simulink model "elevator"  (R2020a)
settings: Solver=VariableStepAuto  StartTime=0.0  StopTime=inf  RelTol=1e-3
PreLoadFcn:
  | slplc.api.loadDataTypes;
undefined symbols (not defined in the file): BOOL, DINT, INT, slplc
libraries: simulink x1
(part 2 of 38)

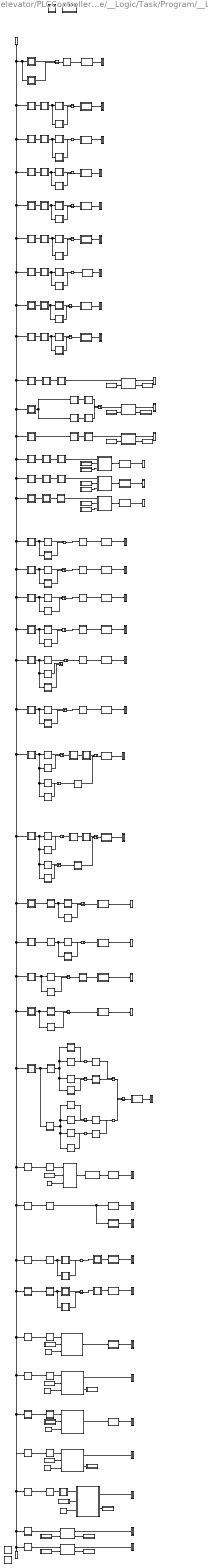
== system elevator/PLCControllerSuite/__Logic/Task/Program/__Logic ==
  note: Increment motor speed by 0.01
  note: Latch motor increase procedure
  note: Initiate motor speed decrease after appropriate sensor is triggered
  note: Trigger motor to increase speed after delay
  note: Indicates when the last direction traveled was up.
  note: Checking for appropriate floor sensor to initiate slow down.
  note: Motor is ON
  note: Motor direction is down
  note: Motor direction is up
  note: Request floor 1
  note: Start/Stop
  note: Request floor 2
  note: Request floor 3
  note: Request elevator to go to floor 2
  note: Memory, to control motor to go down.
  note: Request elevator to go to floor 1
  note: Memory, to control motor to go up.
  note: Request elevator to go to floor 3
  note: Tracck Floor 1
  note: Tracck Floor 2
  note: Tracck Floor 3
  note: Store current position if floor 1
  note: Store current position if floor 2
  note: Store current position if floor 3
  note: TracK Elevator going away or towards Floor 3
  note: TracK Elevator going away or towards Floor 2
  note: TracK Elevator going away or towards Floor 1
  note: Latch motor decrease procedure
  note: Decriment motor speed by 0.01
  note: Set motor speed to 0 when at appropriate floor
  note: Increase speed if less than or equal MAXVEL
  note: Decrease speed if greater than ZERO
  note: Send motor speed out
  note: Send motor speed out
  ADD : Subsystem  Priority=274  TreatAsAtomicUnit=on  mask{PLCBlockType=ADD, PLCPOUType=stdFC}
      mask Help: web([docroot '/plccoder/ref/add' '.html']);
      mask DialogControl PLCBlockTitle Prompt: Add (ADD)
      mask DialogControl PLCBlockDesc Prompt: Add Source A and Source B.
      mask Display: disp('ADD');
  Add Rungs : Subsystem  DisableCoverage=on  TreatAsAtomicUnit=on  mask{PLCRungNumberToAdd=1, PLCBlockType=AddRungs}
      mask prompts: PLCRungNumberToAdd "Rung Number:"
      mask Help: web([docroot '/plccoder/ref/addrungs' '.html']);
      mask DialogControl PLCAddRungs Prompt: Add Rungs
      mask DialogControl PLCRungAddButton Prompt: Add
      mask DialogControl PLCRungAddButton Callback: slplc.callbacks.addLadderRungs(gcb);
      mask Display: disp(sprintf(['Add' newline 'Rungs']));
  Add Single Rung : Subsystem  DisableCoverage=on  TreatAsAtomicUnit=on  mask{PLCRungNumberToAdd=1, PLCBlockType=AddSingleRung}
      settings: OpenFcn=slplc.callbacks.addLadderRungs(gcb);
      mask Help: web([docroot '/plccoder/ref/addsinglerung' '.html']);
      mask DialogControl PLCAddRung Prompt: Add Single Rung
      mask Display: disp(sprintf(['Add' newline '1 Rung']));
  Constant : Constant  Priority=236  Value=0
  Constant1 : Constant  Priority=273  Value=0.01
  Constant2 : Constant  Priority=287  Value=0.01
  Constant3 : Constant  Priority=295  Value=0
  Constant4 : Constant  Priority=266  Value=24
  Constant5 : Constant  Priority=280  Value=0.01
  EQU : Subsystem  Priority=109  TreatAsAtomicUnit=on  mask{PLCBlockType=EQU, PLCPOUType=stdFC}
      mask Help: web([docroot '/plccoder/ref/equ' '.html']);
      mask DialogControl PLCBlockTitle Prompt: Equal To (EQU)
      mask DialogControl PLCBlockDesc Prompt: Test whether Source A is equal to Source B.
      mask Display: disp('EQU');
  EQU1 : Subsystem  Priority=101  TreatAsAtomicUnit=on  mask{PLCBlockType=EQU, PLCPOUType=stdFC}
      mask Help: web([docroot '/plccoder/ref/equ' '.html']);
      mask DialogControl PLCBlockTitle Prompt: Equal To (EQU)
      mask DialogControl PLCBlockDesc Prompt: Test whether Source A is equal to Source B.
      mask Display: disp('EQU');
  EQU2 : Subsystem  Priority=93  TreatAsAtomicUnit=on  mask{PLCBlockType=EQU, PLCPOUType=stdFC}
      mask Help: web([docroot '/plccoder/ref/equ' '.html']);
      mask DialogControl PLCBlockTitle Prompt: Equal To (EQU)
      mask DialogControl PLCBlockDesc Prompt: Test whether Source A is equal to Source B.
      mask Display: disp('EQU');
  EQU3 : Subsystem  Priority=237  TreatAsAtomicUnit=on  mask{PLCBlockType=EQU, PLCPOUType=stdFC}
      mask Help: web([docroot '/plccoder/ref/equ' '.html']);
      mask DialogControl PLCBlockTitle Prompt: Equal To (EQU)
      mask DialogControl PLCBlockDesc Prompt: Test whether Source A is equal to Source B.
      mask Display: disp('EQU');
  GRT : Subsystem  Priority=281  TreatAsAtomicUnit=on  mask{PLCBlockType=GRT, PLCPOUType=stdFC}
      mask Help: web([docroot '/plccoder/ref/grt' '.html']);
      mask DialogControl PLCBlockTitle Prompt: Greater Than (GRT)
      mask DialogControl PLCBlockDesc Prompt: Test whether Source A is greater than Source B.
      mask Display: disp('GRT');
  Junction : Subsystem  Priority=186  DisableCoverage=on  TreatAsAtomicUnit=on  mask{PLCBlockType=Junction, PLCPOUType=BranchJunction}
      mask Help: web([docroot '/plccoder/ref/junction' '.html']);
      mask DialogControl PLCBlockTitle Prompt: Rung Merge Point
      mask DialogControl PLCBlockDesc Prompt: This is the ladder diagram rung merge point.
  Junction1 : Subsystem  Priority=115  DisableCoverage=on  TreatAsAtomicUnit=on  mask{PLCBlockType=Junction, PLCPOUType=BranchJunction}
      mask Help: web([docroot '/plccoder/ref/junction' '.html']);
      mask DialogControl PLCBlockTitle Prompt: Rung Merge Point
      mask DialogControl PLCBlockDesc Prompt: This is the ladder diagram rung merge point.
  Junction10 : Subsystem  Priority=164  DisableCoverage=on  TreatAsAtomicUnit=on  mask{PLCBlockType=Junction, PLCPOUType=BranchJunction}
      mask Help: web([docroot '/plccoder/ref/junction' '.html']);
      mask DialogControl PLCBlockTitle Prompt: Rung Merge Point
      mask DialogControl PLCBlockDesc Prompt: This is the ladder diagram rung merge point.
  Junction11 : Subsystem  Priority=179  DisableCoverage=on  TreatAsAtomicUnit=on  mask{PLCBlockType=Junction, PLCPOUType=BranchJunction}
      mask Help: web([docroot '/plccoder/ref/junction' '.html']);
      mask DialogControl PLCBlockTitle Prompt: Rung Merge Point
      mask DialogControl PLCBlockDesc Prompt: This is the ladder diagram rung merge point.
  Junction12 : Subsystem  Priority=172  DisableCoverage=on  TreatAsAtomicUnit=on  mask{PLCBlockType=Junction, PLCPOUType=BranchJunction}
      mask Help: web([docroot '/plccoder/ref/junction' '.html']);
      mask DialogControl PLCBlockTitle Prompt: Rung Merge Point
      mask DialogControl PLCBlockDesc Prompt: This is the ladder diagram rung merge point.
  Junction13 : Subsystem  Priority=177  DisableCoverage=on  TreatAsAtomicUnit=on  mask{PLCBlockType=Junction, PLCPOUType=BranchJunction}
      mask Help: web([docroot '/plccoder/ref/junction' '.html']);
      mask DialogControl PLCBlockTitle Prompt: Rung Merge Point
      mask DialogControl PLCBlockDesc Prompt: This is the ladder diagram rung merge point.
  Junction14 : Subsystem  Priority=227  DisableCoverage=on  TreatAsAtomicUnit=on  mask{PLCBlockType=Junction, PLCPOUType=BranchJunction}
      mask Help: web([docroot '/plccoder/ref/junction' '.html']);
      mask DialogControl PLCBlockTitle Prompt: Rung Merge Point
      mask DialogControl PLCBlockDesc Prompt: This is the ladder diagram rung merge point.
  Junction15 : Subsystem  Priority=223  DisableCoverage=on  TreatAsAtomicUnit=on  mask{PLCBlockType=Junction, PLCPOUType=BranchJunction}
      mask Help: web([docroot '/plccoder/ref/junction' '.html']);
      mask DialogControl PLCBlockTitle Prompt: Rung Merge Point
      mask DialogControl PLCBlockDesc Prompt: This is the ladder diagram rung merge point.
  Junction16 : Subsystem  Priority=219  DisableCoverage=on  TreatAsAtomicUnit=on  mask{PLCBlockType=Junction, PLCPOUType=BranchJunction}
      mask Help: web([docroot '/plccoder/ref/junction' '.html']);
      mask DialogControl PLCBlockTitle Prompt: Rung Merge Point
      mask DialogControl PLCBlockDesc Prompt: This is the ladder diagram rung merge point.
  Junction17 : Subsystem  Priority=229  DisableCoverage=on  TreatAsAtomicUnit=on  mask{PLCBlockType=Junction, PLCPOUType=BranchJunction}
      mask Help: web([docroot '/plccoder/ref/junction' '.html']);
      mask DialogControl PLCBlockTitle Prompt: Rung Merge Point
      mask DialogControl PLCBlockDesc Prompt: This is the ladder diagram rung merge point.
  Junction18 : Subsystem  Priority=193  DisableCoverage=on  TreatAsAtomicUnit=on  mask{PLCBlockType=Junction, PLCPOUType=BranchJunction}
      mask Help: web([docroot '/plccoder/ref/junction' '.html']);
      mask DialogControl PLCBlockTitle Prompt: Rung Merge Point
      mask DialogControl PLCBlockDesc Prompt: This is the ladder diagram rung merge point.
  Junction19 : Subsystem  Priority=213  DisableCoverage=on  TreatAsAtomicUnit=on  mask{PLCBlockType=Junction, PLCPOUType=BranchJunction}
      mask Help: web([docroot '/plccoder/ref/junction' '.html']);
      mask DialogControl PLCBlockTitle Prompt: Rung Merge Point
      mask DialogControl PLCBlockDesc Prompt: This is the ladder diagram rung merge point.
  Junction2 : Subsystem  Priority=122  DisableCoverage=on  TreatAsAtomicUnit=on  mask{PLCBlockType=Junction, PLCPOUType=BranchJunction}
      mask Help: web([docroot '/plccoder/ref/junction' '.html']);
      mask DialogControl PLCBlockTitle Prompt: Rung Merge Point
      mask DialogControl PLCBlockDesc Prompt: This is the ladder diagram rung merge point.
  Junction20 : Subsystem  Priority=4  DisableCoverage=on  TreatAsAtomicUnit=on  mask{PLCBlockType=Junction, PLCPOUType=BranchJunction}
      mask Help: web([docroot '/plccoder/ref/junction' '.html']);
      mask DialogControl PLCBlockTitle Prompt: Rung Merge Point
      mask DialogControl PLCBlockDesc Prompt: This is the ladder diagram rung merge point.
  Junction21 : Subsystem  Priority=217  DisableCoverage=on  TreatAsAtomicUnit=on  mask{PLCBlockType=Junction, PLCPOUType=BranchJunction}
      mask Help: web([docroot '/plccoder/ref/junction' '.html']);
      mask DialogControl PLCBlockTitle Prompt: Rung Merge Point
      mask DialogControl PLCBlockDesc Prompt: This is the ladder diagram rung merge point.
  Junction22 : Subsystem  Priority=19  DisableCoverage=on  TreatAsAtomicUnit=on  mask{PLCBlockType=Junction, PLCPOUType=BranchJunction}
      mask Help: web([docroot '/plccoder/ref/junction' '.html']);
      mask DialogControl PLCBlockTitle Prompt: Rung Merge Point
      mask DialogControl PLCBlockDesc Prompt: This is the ladder diagram rung merge point.
  Junction23 : Subsystem  Priority=26  DisableCoverage=on  TreatAsAtomicUnit=on  mask{PLCBlockType=Junction, PLCPOUType=BranchJunction}
      mask Help: web([docroot '/plccoder/ref/junction' '.html']);
      mask DialogControl PLCBlockTitle Prompt: Rung Merge Point
      mask DialogControl PLCBlockDesc Prompt: This is the ladder diagram rung merge point.
  Junction24 : Subsystem  Priority=76  DisableCoverage=on  TreatAsAtomicUnit=on  mask{PLCBlockType=Junction, PLCPOUType=BranchJunction}
      mask Help: web([docroot '/plccoder/ref/junction' '.html']);
      mask DialogControl PLCBlockTitle Prompt: Rung Merge Point
      mask DialogControl PLCBlockDesc Prompt: This is the ladder diagram rung merge point.
  Junction25 : Subsystem  Priority=54  DisableCoverage=on  TreatAsAtomicUnit=on  mask{PLCBlockType=Junction, PLCPOUType=BranchJunction}
      mask Help: web([docroot '/plccoder/ref/junction' '.html']);
      mask DialogControl PLCBlockTitle Prompt: Rung Merge Point
      mask DialogControl PLCBlockDesc Prompt: This is the ladder diagram rung merge point.
  Junction26 : Subsystem  Priority=40  DisableCoverage=on  TreatAsAtomicUnit=on  mask{PLCBlockType=Junction, PLCPOUType=BranchJunction}
      mask Help: web([docroot '/plccoder/ref/junction' '.html']);
      mask DialogControl PLCBlockTitle Prompt: Rung Merge Point
      mask DialogControl PLCBlockDesc Prompt: This is the ladder diagram rung merge point.
  Junction27 : Subsystem  Priority=61  DisableCoverage=on  TreatAsAtomicUnit=on  mask{PLCBlockType=Junction, PLCPOUType=BranchJunction}
      mask Help: web([docroot '/plccoder/ref/junction' '.html']);
      mask DialogControl PLCBlockTitle Prompt: Rung Merge Point
      mask DialogControl PLCBlockDesc Prompt: This is the ladder diagram rung merge point.
  Junction28 : Subsystem  Priority=47  DisableCoverage=on  TreatAsAtomicUnit=on  mask{PLCBlockType=Junction, PLCPOUType=BranchJunction}
      mask Help: web([docroot '/plccoder/ref/junction' '.html']);
      mask DialogControl PLCBlockTitle Prompt: Rung Merge Point
      mask DialogControl PLCBlockDesc Prompt: This is the ladder diagram rung merge point.
  Junction29 : Subsystem  Priority=206  DisableCoverage=on  TreatAsAtomicUnit=on  mask{PLCBlockType=Junction, PLCPOUType=BranchJunction}
      mask Help: web([docroot '/plccoder/ref/junction' '.html']);
      mask DialogControl PLCBlockTitle Prompt: Rung Merge Point
      mask DialogControl PLCBlockDesc Prompt: This is the ladder diagram rung merge point.
  Junction3 : Subsystem  Priority=129  DisableCoverage=on  TreatAsAtomicUnit=on  mask{PLCBlockType=Junction, PLCPOUType=BranchJunction}
      mask Help: web([docroot '/plccoder/ref/junction' '.html']);
      mask DialogControl PLCBlockTitle Prompt: Rung Merge Point
      mask DialogControl PLCBlockDesc Prompt: This is the ladder diagram rung merge point.
  Junction30 : Subsystem  Priority=230  DisableCoverage=on  TreatAsAtomicUnit=on  mask{PLCBlockType=Junction, PLCPOUType=BranchJunction}
      mask Help: web([docroot '/plccoder/ref/junction' '.html']);
      mask DialogControl PLCBlockTitle Prompt: Rung Merge Point
      mask DialogControl PLCBlockDesc Prompt: This is the ladder diagram rung merge point.
  Junction31 : Subsystem  Priority=199  DisableCoverage=on  TreatAsAtomicUnit=on  mask{PLCBlockType=Junction, PLCPOUType=BranchJunction}
      mask Help: web([docroot '/plccoder/ref/junction' '.html']);
      mask DialogControl PLCBlockTitle Prompt: Rung Merge Point
      mask DialogControl PLCBlockDesc Prompt: This is the ladder diagram rung merge point.
  Junction32 : Subsystem  Priority=33  DisableCoverage=on  TreatAsAtomicUnit=on  mask{PLCBlockType=Junction, PLCPOUType=BranchJunction}
      mask Help: web([docroot '/plccoder/ref/junction' '.html']);
      mask DialogControl PLCBlockTitle Prompt: Rung Merge Point
      mask DialogControl PLCBlockDesc Prompt: This is the ladder diagram rung merge point.
  Junction33 : Subsystem  Priority=12  DisableCoverage=on  TreatAsAtomicUnit=on  mask{PLCBlockType=Junction, PLCPOUType=BranchJunction}
      mask Help: web([docroot '/plccoder/ref/junction' '.html']);
      mask DialogControl PLCBlockTitle Prompt: Rung Merge Point
      mask DialogControl PLCBlockDesc Prompt: This is the ladder diagram rung merge point.
  Junction34 : Subsystem  Priority=251  DisableCoverage=on  TreatAsAtomicUnit=on  mask{PLCBlockType=Junction, PLCPOUType=BranchJunction}
      mask Help: web([docroot '/plccoder/ref/junction' '.html']);
      mask DialogControl PLCBlockTitle Prompt: Rung Merge Point
      mask DialogControl PLCBlockDesc Prompt: This is the ladder diagram rung merge point.
  Junction35 : Subsystem  Priority=259  DisableCoverage=on  TreatAsAtomicUnit=on  mask{PLCBlockType=Junction, PLCPOUType=BranchJunction}
      mask Help: web([docroot '/plccoder/ref/junction' '.html']);
      mask DialogControl PLCBlockTitle Prompt: Rung Merge Point
      mask DialogControl PLCBlockDesc Prompt: This is the ladder diagram rung merge point.
  Junction4 : Subsystem  Priority=136  DisableCoverage=on  TreatAsAtomicUnit=on  mask{PLCBlockType=Junction, PLCPOUType=BranchJunction}
      mask Help: web([docroot '/plccoder/ref/junction' '.html']);
      mask DialogControl PLCBlockTitle Prompt: Rung Merge Point
      mask DialogControl PLCBlockDesc Prompt: This is the ladder diagram rung merge point.
  Junction5 : Subsystem  Priority=145  DisableCoverage=on  TreatAsAtomicUnit=on  mask{PLCBlockType=Junction, PLCPOUType=BranchJunction}
      mask Help: web([docroot '/plccoder/ref/junction' '.html']);
      mask DialogControl PLCBlockTitle Prompt: Rung Merge Point
      mask DialogControl PLCBlockDesc Prompt: This is the ladder diagram rung merge point.
  Junction6 : Subsystem  Priority=144  DisableCoverage=on  TreatAsAtomicUnit=on  mask{PLCBlockType=Junction, PLCPOUType=BranchJunction}
      mask Help: web([docroot '/plccoder/ref/junction' '.html']);
      mask DialogControl PLCBlockTitle Prompt: Rung Merge Point
      mask DialogControl PLCBlockDesc Prompt: This is the ladder diagram rung merge point.
  Junction7 : Subsystem  Priority=152  DisableCoverage=on  TreatAsAtomicUnit=on  mask{PLCBlockType=Junction, PLCPOUType=BranchJunction}
      mask Help: web([docroot '/plccoder/ref/junction' '.html']);
      mask DialogControl PLCBlockTitle Prompt: Rung Merge Point
      mask DialogControl PLCBlockDesc Prompt: This is the ladder diagram rung merge point.
  Junction8 : Subsystem  Priority=159  DisableCoverage=on  TreatAsAtomicUnit=on  mask{PLCBlockType=Junction, PLCPOUType=BranchJunction}
      mask Help: web([docroot '/plccoder/ref/junction' '.html']);
      mask DialogControl PLCBlockTitle Prompt: Rung Merge Point
      mask DialogControl PLCBlockDesc Prompt: This is the ladder diagram rung merge point.
  Junction9 : Subsystem  Priority=166  DisableCoverage=on  TreatAsAtomicUnit=on  mask{PLCBlockType=Junction, PLCPOUType=BranchJunction}
      mask Help: web([docroot '/plccoder/ref/junction' '.html']);
      mask DialogControl PLCBlockTitle Prompt: Rung Merge Point
      mask DialogControl PLCBlockDesc Prompt: This is the ladder diagram rung merge point.
  LEQ : Subsystem  Priority=267  TreatAsAtomicUnit=on  mask{PLCBlockType=LEQ, PLCPOUType=stdFC}
      mask Help: web([docroot '/plccoder/ref/leq' '.html']);
      mask DialogControl PLCBlockTitle Prompt: Less Than or Equal To (LEQ)
      mask DialogControl PLCBlockDesc Prompt: Test whether Source A is less than or equal to Source B.
      mask Display: disp('LEQ');
  MOV : Subsystem  Priority=301  TreatAsAtomicUnit=on  mask{PLCBlockType=MOV, PLCPOUType=stdFC}
      mask Help: web([docroot '/plccoder/ref/mov' '.html']);
      mask DialogControl PLCBlockTitle Prompt: Move (MOV)
      mask DialogControl PLCBlockDesc Prompt: Move a copy of the Source to the Destination. The Source remains unchanged.
      mask Display: disp('MOV');
  MOV1 : Subsystem  Priority=85  TreatAsAtomicUnit=on  mask{PLCBlockType=MOV, PLCPOUType=stdFC}
      mask Help: web([docroot '/plccoder/ref/mov' '.html']);
      mask DialogControl PLCBlockTitle Prompt: Move (MOV)
      mask DialogControl PLCBlockDesc Prompt: Move a copy of the Source to the Destination. The Source remains unchanged.
      mask Display: disp('MOV');
  MOV2 : Subsystem  Priority=78  TreatAsAtomicUnit=on  mask{PLCBlockType=MOV, PLCPOUType=stdFC}
      mask Help: web([docroot '/plccoder/ref/mov' '.html']);
      mask DialogControl PLCBlockTitle Prompt: Move (MOV)
      mask DialogControl PLCBlockDesc Prompt: Move a copy of the Source to the Destination. The Source remains unchanged.
      mask Display: disp('MOV');
  MOV3 : Subsystem  Priority=68  TreatAsAtomicUnit=on  mask{PLCBlockType=MOV, PLCPOUType=stdFC}
      mask Help: web([docroot '/plccoder/ref/mov' '.html']);
      mask DialogControl PLCBlockTitle Prompt: Move (MOV)
      mask DialogControl PLCBlockDesc Prompt: Move a copy of the Source to the Destination. The Source remains unchanged.
      mask Display: disp('MOV');
  MOV4 : Subsystem  Priority=306  TreatAsAtomicUnit=on  mask{PLCBlockType=MOV, PLCPOUType=stdFC}
      mask Help: web([docroot '/plccoder/ref/mov' '.html']);
      mask DialogControl PLCBlockTitle Prompt: Move (MOV)
      mask DialogControl PLCBlockDesc Prompt: Move a copy of the Source to the Destination. The Source remains unchanged.
      mask Display: disp('MOV');
  MUL : Subsystem  Priority=296  TreatAsAtomicUnit=on  mask{PLCBlockType=MUL, PLCPOUType=stdFC}
      mask Help: web([docroot '/plccoder/ref/mul' '.html']);
      mask DialogControl PLCBlockTitle Prompt: Multiply (MUL)
      mask DialogControl PLCBlockDesc Prompt: Multiply Source A with Source B.
      mask Display: disp('MUL');
  OTE : Subsystem  Priority=6  TreatAsAtomicUnit=on  mask{PLCOperandTag=StartHold, PLCBlockType=OTE, PLCPOUType=Coil, PLCOperandExpression=xxx_PLC_VAR_StartHold}
      mask prompts: PLCOperandTag "Operand Tag:"
      mask init:
      | slplc.callbacks.initInstruction(gcb);
      settings: AttributesFormatString=%<PLCOperandTag>
      mask Help: web([docroot '/plccoder/ref/ote' '.html']);
      mask DialogControl PLCBlockTitle Prompt: Output Energize (OTE)
  OTE1 : Subsystem  Priority=117  TreatAsAtomicUnit=on  mask{PLCOperandTag=F1PBHold, PLCBlockType=OTE, PLCPOUType=Coil, PLCOperandExpression=xxx_PLC_VAR_F1PBHold}
      mask prompts: PLCOperandTag "Operand Tag:"
      mask init:
      | slplc.callbacks.initInstruction(gcb);
      settings: AttributesFormatString=%<PLCOperandTag>
      mask Help: web([docroot '/plccoder/ref/ote' '.html']);
      mask DialogControl PLCBlockTitle Prompt: Output Energize (OTE)
  OTE10 : Subsystem  Priority=180  TreatAsAtomicUnit=on  mask{PLCOperandTag=MemoryGoDown, PLCBlockType=OTE, PLCPOUType=Coil, PLCOperandExpression=xxx_PLC_VAR_MemoryGoDown}
      mask prompts: PLCOperandTag "Operand Tag:"
      mask init:
      | slplc.callbacks.initInstruction(gcb);
      settings: AttributesFormatString=%<PLCOperandTag>
      mask Help: web([docroot '/plccoder/ref/ote' '.html']);
      mask DialogControl PLCBlockTitle Prompt: Output Energize (OTE)
  OTE11 : Subsystem  Priority=239  TreatAsAtomicUnit=on  mask{PLCOperandTag=RMPUPTRG, PLCBlockType=OTE, PLCPOUType=Coil, PLCOperandExpression=xxx_PLC_VAR_RMPUPTRG}
      mask prompts: PLCOperandTag "Operand Tag:"
      mask init:
      | slplc.callbacks.initInstruction(gcb);
      settings: AttributesFormatString=%<PLCOperandTag>
      mask Help: web([docroot '/plccoder/ref/ote' '.html']);
      mask DialogControl PLCBlockTitle Prompt: Output Energize (OTE)
  OTE12 : Subsystem  Priority=253  TreatAsAtomicUnit=on  mask{PLCOperandTag=RMPUP, PLCBlockType=OTE, PLCPOUType=Coil, PLCOperandExpression=xxx_PLC_VAR_RMPUP}
      mask prompts: PLCOperandTag "Operand Tag:"
      mask init:
      | slplc.callbacks.initInstruction(gcb);
      settings: AttributesFormatString=%<PLCOperandTag>
      mask Help: web([docroot '/plccoder/ref/ote' '.html']);
      mask DialogControl PLCBlockTitle Prompt: Output Energize (OTE)
  OTE13 : Subsystem  Priority=261  TreatAsAtomicUnit=on  mask{PLCOperandTag=RMPDN, PLCBlockType=OTE, PLCPOUType=Coil, PLCOperandExpression=xxx_PLC_VAR_RMPDN}
      mask prompts: PLCOperandTag "Operand Tag:"
      mask init:
      | slplc.callbacks.initInstruction(gcb);
      settings: AttributesFormatString=%<PLCOperandTag>
      mask Help: web([docroot '/plccoder/ref/ote' '.html']);
      mask DialogControl PLCBlockTitle Prompt: Output Energize (OTE)
  OTE14 : Subsystem  Priority=243  TreatAsAtomicUnit=on  mask{PLCOperandTag=RMPUPKIL, PLCBlockType=OTE, PLCPOUType=Coil, PLCOperandExpression=xxx_PLC_VAR_RMPUPKIL}
      mask prompts: PLCOperandTag "Operand Tag:"
      mask init:
      | slplc.callbacks.initInstruction(gcb);
      settings: AttributesFormatString=%<PLCOperandTag>
      mask Help: web([docroot '/plccoder/ref/ote' '.html']);
      mask DialogControl PLCBlockTitle Prompt: Output Energize (OTE)
  OTE15 : Subsystem  Priority=62  TreatAsAtomicUnit=on  mask{PLCOperandTag=TempS1HUp, PLCBlockType=OTE, PLCPOUType=Coil, PLCOperandExpression=xxx_PLC_VAR_TempS1HUp}
      mask prompts: PLCOperandTag "Operand Tag:"
      mask init:
      | slplc.callbacks.initInstruction(gcb);
      settings: AttributesFormatString=%<PLCOperandTag>
      mask Help: web([docroot '/plccoder/ref/ote' '.html']);
      mask DialogControl PLCBlockTitle Prompt: Output Energize (OTE)
  OTE16 : Subsystem  Priority=48  TreatAsAtomicUnit=on  mask{PLCOperandTag=TempS2LUp, PLCBlockType=OTE, PLCPOUType=Coil, PLCOperandExpression=xxx_PLC_VAR_TempS2LUp}
      mask prompts: PLCOperandTag "Operand Tag:"
      mask init:
      | slplc.callbacks.initInstruction(gcb);
      settings: AttributesFormatString=%<PLCOperandTag>
      mask Help: web([docroot '/plccoder/ref/ote' '.html']);
      mask DialogControl PLCBlockTitle Prompt: Output Energize (OTE)
  OTE17 : Subsystem  Priority=20  TreatAsAtomicUnit=on  mask{PLCOperandTag=TempS3LUp, PLCBlockType=OTE, PLCPOUType=Coil, PLCOperandExpression=xxx_PLC_VAR_TempS3LUp}
      mask prompts: PLCOperandTag "Operand Tag:"
      mask init:
      | slplc.callbacks.initInstruction(gcb);
      settings: AttributesFormatString=%<PLCOperandTag>
      mask Help: web([docroot '/plccoder/ref/ote' '.html']);
      mask DialogControl PLCBlockTitle Prompt: Output Energize (OTE)
  OTE18 : Subsystem  Priority=27  TreatAsAtomicUnit=on  mask{PLCOperandTag=TempS2HDown, PLCBlockType=OTE, PLCPOUType=Coil, PLCOperandExpression=xxx_PLC_VAR_TempS2HDown}
      mask prompts: PLCOperandTag "Operand Tag:"
      mask init:
      | slplc.callbacks.initInstruction(gcb);
      settings: AttributesFormatString=%<PLCOperandTag>
      mask Help: web([docroot '/plccoder/ref/ote' '.html']);
      mask DialogControl PLCBlockTitle Prompt: Output Energize (OTE)
  OTE19 : Subsystem  Priority=41  TreatAsAtomicUnit=on  mask{PLCOperandTag=TempS2LDown, PLCBlockType=OTE, PLCPOUType=Coil, PLCOperandExpression=xxx_PLC_VAR_TempS2LDown}
      mask prompts: PLCOperandTag "Operand Tag:"
      mask init:
      | slplc.callbacks.initInstruction(gcb);
      settings: AttributesFormatString=%<PLCOperandTag>
      mask Help: web([docroot '/plccoder/ref/ote' '.html']);
      mask DialogControl PLCBlockTitle Prompt: Output Energize (OTE)
  OTE2 : Subsystem  Priority=124  TreatAsAtomicUnit=on  mask{PLCOperandTag=F2PBHold, PLCBlockType=OTE, PLCPOUType=Coil, PLCOperandExpression=xxx_PLC_VAR_F2PBHold}
      mask prompts: PLCOperandTag "Operand Tag:"
      mask init:
      | slplc.callbacks.initInstruction(gcb);
      settings: AttributesFormatString=%<PLCOperandTag>
      mask Help: web([docroot '/plccoder/ref/ote' '.html']);
      mask DialogControl PLCBlockTitle Prompt: Output Energize (OTE)
  OTE20 : Subsystem  Priority=55  TreatAsAtomicUnit=on  mask{PLCOperandTag=TempS1HDown, PLCBlockType=OTE, PLCPOUType=Coil, PLCOperandExpression=xxx_PLC_VAR_TempS1HDown}
      mask prompts: PLCOperandTag "Operand Tag:"
      mask init:
      | slplc.callbacks.initInstruction(gcb);
      settings: AttributesFormatString=%<PLCOperandTag>
      mask Help: web([docroot '/plccoder/ref/ote' '.html']);
      mask DialogControl PLCBlockTitle Prompt: Output Energize (OTE)
  OTE21 : Subsystem  Priority=34  TreatAsAtomicUnit=on  mask{PLCOperandTag=TempS2HUp, PLCBlockType=OTE, PLCPOUType=Coil, PLCOperandExpression=xxx_PLC_VAR_TempS2HUp}
      mask prompts: PLCOperandTag "Operand Tag:"
      mask init:
      | slplc.callbacks.initInstruction(gcb);
      settings: AttributesFormatString=%<PLCOperandTag>
      mask Help: web([docroot '/plccoder/ref/ote' '.html']);
      mask DialogControl PLCBlockTitle Prompt: Output Energize (OTE)
  OTE22 : Subsystem  Priority=13  TreatAsAtomicUnit=on  mask{PLCOperandTag=TempS3LDown, PLCBlockType=OTE, PLCPOUType=Coil, PLCOperandExpression=xxx_PLC_VAR_TempS3LDown}
      mask prompts: PLCOperandTag "Operand Tag:"
      mask init:
      | slplc.callbacks.initInstruction(gcb);
      settings: AttributesFormatString=%<PLCOperandTag>
      mask Help: web([docroot '/plccoder/ref/ote' '.html']);
      mask DialogControl PLCBlockTitle Prompt: Output Energize (OTE)
  OTE23 : Subsystem  Priority=110  TreatAsAtomicUnit=on  mask{PLCOperandTag=AtFloor1, PLCBlockType=OTE, PLCPOUType=Coil, PLCOperandExpression=xxx_PLC_VAR_AtFloor1}
      mask prompts: PLCOperandTag "Operand Tag:"
      mask init:
      | slplc.callbacks.initInstruction(gcb);
      settings: AttributesFormatString=%<PLCOperandTag>
      mask Help: web([docroot '/plccoder/ref/ote' '.html']);
      mask DialogControl PLCBlockTitle Prompt: Output Energize (OTE)
  OTE24 : Subsystem  Priority=102  TreatAsAtomicUnit=on  mask{PLCOperandTag=AtFloor2, PLCBlockType=OTE, PLCPOUType=Coil, PLCOperandExpression=xxx_PLC_VAR_AtFloor2}
      mask prompts: PLCOperandTag "Operand Tag:"
      mask init:
      | slplc.callbacks.initInstruction(gcb);
      settings: AttributesFormatString=%<PLCOperandTag>
      mask Help: web([docroot '/plccoder/ref/ote' '.html']);
      mask DialogControl PLCBlockTitle Prompt: Output Energize (OTE)
  OTE25 : Subsystem  Priority=94  TreatAsAtomicUnit=on  mask{PLCOperandTag=AtFloor3, PLCBlockType=OTE, PLCPOUType=Coil, PLCOperandExpression=xxx_PLC_VAR_AtFloor3}
      mask prompts: PLCOperandTag "Operand Tag:"
      mask init:
      | slplc.callbacks.initInstruction(gcb);
      settings: AttributesFormatString=%<PLCOperandTag>
      mask Help: web([docroot '/plccoder/ref/ote' '.html']);
      mask DialogControl PLCBlockTitle Prompt: Output Energize (OTE)
  OTE26 : Subsystem  Priority=187  TreatAsAtomicUnit=on  mask{PLCOperandTag=GOINGUP, PLCBlockType=OTE, PLCPOUType=Coil, PLCOperandExpression=xxx_PLC_VAR_GOINGUP}
      mask prompts: PLCOperandTag "Operand Tag:"
      mask init:
      | slplc.callbacks.initInstruction(gcb);
      settings: AttributesFormatString=%<PLCOperandTag>
      mask Help: web([docroot '/plccoder/ref/ote' '.html']);
      mask DialogControl PLCBlockTitle Prompt: Output Energize (OTE)
  OTE27 : Subsystem  Priority=194  TreatAsAtomicUnit=on  mask{PLCOperandTag=GOINGDN, PLCBlockType=OTE, PLCPOUType=Coil, PLCOperandExpression=xxx_PLC_VAR_GOINGDN}
      mask prompts: PLCOperandTag "Operand Tag:"
      mask init:
      | slplc.callbacks.initInstruction(gcb);
      settings: AttributesFormatString=%<PLCOperandTag>
      mask Help: web([docroot '/plccoder/ref/ote' '.html']);
      mask DialogControl PLCBlockTitle Prompt: Output Energize (OTE)
  OTE28 : Subsystem  Priority=207  TreatAsAtomicUnit=on  mask{PLCOperandTag=MTRON, PLCBlockType=OTE, PLCPOUType=Coil, PLCOperandExpression=xxx_PLC_VAR_MTRON}
      mask prompts: PLCOperandTag "Operand Tag:"
      mask init:
      | slplc.callbacks.initInstruction(gcb);
      settings: AttributesFormatString=%<PLCOperandTag>
      mask Help: web([docroot '/plccoder/ref/ote' '.html']);
      mask DialogControl PLCBlockTitle Prompt: Output Energize (OTE)
  OTE29 : Subsystem  Priority=245  TreatAsAtomicUnit=on  mask{PLCOperandTag=RMPDNTRG, PLCBlockType=OTE, PLCPOUType=Coil, PLCOperandExpression=xxx_PLC_VAR_RMPDNTRG}
      mask prompts: PLCOperandTag "Operand Tag:"
      mask init:
      | slplc.callbacks.initInstruction(gcb);
      settings: AttributesFormatString=%<PLCOperandTag>
      mask Help: web([docroot '/plccoder/ref/ote' '.html']);
      mask DialogControl PLCBlockTitle Prompt: Output Energize (OTE)
  OTE3 : Subsystem  Priority=131  TreatAsAtomicUnit=on  mask{PLCOperandTag=F3PBHold, PLCBlockType=OTE, PLCPOUType=Coil, PLCOperandExpression=xxx_PLC_VAR_F3PBHold}
      mask prompts: PLCOperandTag "Operand Tag:"
      mask init:
      | slplc.callbacks.initInstruction(gcb);
      settings: AttributesFormatString=%<PLCOperandTag>
      mask Help: web([docroot '/plccoder/ref/ote' '.html']);
      mask DialogControl PLCBlockTitle Prompt: Output Energize (OTE)
  OTE30 : Subsystem  Priority=268  TreatAsAtomicUnit=on  mask{PLCOperandTag=INCSPD, PLCBlockType=OTE, PLCPOUType=Coil, PLCOperandExpression=xxx_PLC_VAR_INCSPD}
      mask prompts: PLCOperandTag "Operand Tag:"
      mask init:
      | slplc.callbacks.initInstruction(gcb);
      settings: AttributesFormatString=%<PLCOperandTag>
      mask Help: web([docroot '/plccoder/ref/ote' '.html']);
      mask DialogControl PLCBlockTitle Prompt: Output Energize (OTE)
  OTE31 : Subsystem  Priority=282  TreatAsAtomicUnit=on  mask{PLCOperandTag=DECSPD, PLCBlockType=OTE, PLCPOUType=Coil, PLCOperandExpression=xxx_PLC_VAR_DECSPD}
      mask prompts: PLCOperandTag "Operand Tag:"
      mask init:
      | slplc.callbacks.initInstruction(gcb);
      settings: AttributesFormatString=%<PLCOperandTag>
      mask Help: web([docroot '/plccoder/ref/ote' '.html']);
      mask DialogControl PLCBlockTitle Prompt: Output Energize (OTE)
  OTE4 : Subsystem  Priority=138  TreatAsAtomicUnit=on  mask{PLCOperandTag=F1UpBHold, PLCBlockType=OTE, PLCPOUType=Coil, PLCOperandExpression=xxx_PLC_VAR_F1UpBHold}
      mask prompts: PLCOperandTag "Operand Tag:"
      mask init:
      | slplc.callbacks.initInstruction(gcb);
      settings: AttributesFormatString=%<PLCOperandTag>
      mask Help: web([docroot '/plccoder/ref/ote' '.html']);
      mask DialogControl PLCBlockTitle Prompt: Output Energize (OTE)
  OTE5 : Subsystem  Priority=147  TreatAsAtomicUnit=on  mask{PLCOperandTag=F2UpDownBHold, PLCBlockType=OTE, PLCPOUType=Coil, PLCOperandExpression=xxx_PLC_VAR_F2UpDownBHold}
      mask prompts: PLCOperandTag "Operand Tag:"
      mask init:
      | slplc.callbacks.initInstruction(gcb);
      settings: AttributesFormatString=%<PLCOperandTag>
      mask Help: web([docroot '/plccoder/ref/ote' '.html']);
      mask DialogControl PLCBlockTitle Prompt: Output Energize (OTE)
  OTE6 : Subsystem  Priority=154  TreatAsAtomicUnit=on  mask{PLCOperandTag=F3DownBHold, PLCBlockType=OTE, PLCPOUType=Coil, PLCOperandExpression=xxx_PLC_VAR_F3DownBHold}
      mask prompts: PLCOperandTag "Operand Tag:"
      mask init:
      | slplc.callbacks.initInstruction(gcb);
      settings: AttributesFormatString=%<PLCOperandTag>
      mask Help: web([docroot '/plccoder/ref/ote' '.html']);
      mask DialogControl PLCBlockTitle Prompt: Output Energize (OTE)
  OTE7 : Subsystem  Priority=231  TreatAsAtomicUnit=on  mask{PLCOperandTag=SENCHK, PLCBlockType=OTE, PLCPOUType=Coil, PLCOperandExpression=xxx_PLC_VAR_SENCHK}
      mask prompts: PLCOperandTag "Operand Tag:"
      mask init:
      | slplc.callbacks.initInstruction(gcb);
      settings: AttributesFormatString=%<PLCOperandTag>
      mask Help: web([docroot '/plccoder/ref/ote' '.html']);
      mask DialogControl PLCBlockTitle Prompt: Output Energize (OTE)
  OTE8 : Subsystem  Priority=201  TreatAsAtomicUnit=on  mask{PLCOperandTag=LSTDIRUP, PLCBlockType=OTE, PLCPOUType=Coil, PLCOperandExpression=xxx_PLC_VAR_LSTDIRUP}
      mask prompts: PLCOperandTag "Operand Tag:"
      mask init:
      | slplc.callbacks.initInstruction(gcb);
      settings: AttributesFormatString=%<PLCOperandTag>
      mask Help: web([docroot '/plccoder/ref/ote' '.html']);
      mask DialogControl PLCBlockTitle Prompt: Output Energize (OTE)
  OTE9 : Subsystem  Priority=167  TreatAsAtomicUnit=on  mask{PLCOperandTag=MemoryGoUp, PLCBlockType=OTE, PLCPOUType=Coil, PLCOperandExpression=xxx_PLC_VAR_MemoryGoUp}
      mask prompts: PLCOperandTag "Operand Tag:"
      mask init:
      | slplc.callbacks.initInstruction(gcb);
      settings: AttributesFormatString=%<PLCOperandTag>
      mask Help: web([docroot '/plccoder/ref/ote' '.html']);
      mask DialogControl PLCBlockTitle Prompt: Output Energize (OTE)
  Power Rail Start : Subsystem  Priority=1  DisableCoverage=on  TreatAsAtomicUnit=on  mask{PLCBlockType=PowerRailStart}
      mask Help: web([docroot '/plccoder/ref/powerrailstart' '.html']);
      mask DialogControl PLCBlockTitle Prompt: Power Rail Start
      mask DialogControl PLCBlockDesc Prompt: This is the ladder diagram left power rail start block.
  Power Rail Terminal : Subsystem  DisableCoverage=on  TreatAsAtomicUnit=on  mask{PLCBlockType=PowerRailTerminal}
      mask Help: web([docroot '/plccoder/ref/powerrailterminal' '.html']);
      mask DialogControl PLCBlockTitle Prompt: Power Rail Terminal
      mask DialogControl PLCBlockDesc Prompt: This is the ladder diagram left power rail terminal block.
  Program Variables : Subsystem  Tag=ProgramVariableSS  DisableCoverage=on  TreatAsAtomicUnit=on  mask{PLCVarAtFloor1Name=AtFloor1, PLCVarAtFloor1Scope=Local, PLCVarAtFloor1PortType=Hidden, PLCVarAtFloor1PortIndex=59, PLCVarAtFloor1DataType=BOOL, PLCVarAtFloor1Size=1, PLCVarAtFloor1InitialValue=false, PLCVarAtFloor1ToDelete=off, PLCVarAtFloor2Name=AtFloor2, PLCVarAtFloor2Scope=Local, PLCVarAtFloor2PortType=Hidden, PLCVarAtFloor2PortIndex=59, PLCVarAtFloor2DataType=BOOL, PLCVarAtFloor2Size=1, PLCVarAtFloor2InitialValue=false, PLCVarAtFloor2ToDelete=off, PLCVarAtFloor3Name=AtFloor3, PLCVarAtFloor3Scope=Local, PLCVarAtFloor3PortType=Hidden, PLCVarAtFloor3PortIndex=59, PLCVarAtFloor3DataType=BOOL, PLCVarAtFloor3Size=1, PLCVarAtFloor3InitialValue=false, PLCVarAtFloor3ToDelete=off, PLCVarCurrent_floorName=Current_floor, PLCVarCurrent_floorScope=Local, PLCVarCurrent_floorPortType=Hidden, PLCVarCurrent_floorPortIndex=59, PLCVarCurrent_floorDataType=DINT, PLCVarCurrent_floorSize=1, PLCVarCurrent_floorInitialValue=1, PLCVarCurrent_floorToDelete=off, PLCVarDECSPDName=DECSPD, PLCVarDECSPDScope=Local, PLCVarDECSPDPortType=Hidden, PLCVarDECSPDPortIndex=59, PLCVarDECSPDDataType=BOOL, PLCVarDECSPDSize=1, PLCVarDECSPDInitialValue=false, PLCVarDECSPDToDelete=off, PLCVarF1PBHoldName=F1PBHold, PLCVarF1PBHoldScope=Local, PLCVarF1PBHoldPortType=Hidden, PLCVarF1PBHoldPortIndex=59, PLCVarF1PBHoldDataType=BOOL, PLCVarF1PBHoldSize=1, PLCVarF1PBHoldInitialValue=false, PLCVarF1PBHoldToDelete=off, PLCVarF1UpBHoldName=F1UpBHold, PLCVarF1UpBHoldScope=Local, PLCVarF1UpBHoldPortType=Hidden, PLCVarF1UpBHoldPortIndex=59, PLCVarF1UpBHoldDataType=BOOL, PLCVarF1UpBHoldSize=1, PLCVarF1UpBHoldInitialValue=false, PLCVarF1UpBHoldToDelete=off, PLCVarF2PBHoldName=F2PBHold, PLCVarF2PBHoldScope=Local, PLCVarF2PBHoldPortType=Hidden, PLCVarF2PBHoldPortIndex=59, PLCVarF2PBHoldDataType=BOOL, PLCVarF2PBHoldSize=1, PLCVarF2PBHoldInitialValue=false, PLCVarF2PBHoldToDelete=off, PLCVarF2UpDownBHoldName=F2UpDownBHold, PLCVarF2UpDownBHoldScope=Local, PLCVarF2UpDownBHoldPortType=Hidden, PLCVarF2UpDownBHoldPortIndex=59, PLCVarF2UpDownBHoldDataType=BOOL, PLCVarF2UpDownBHoldSize=1, PLCVarF2UpDownBHoldInitialValue=false, PLCVarF2UpDownBHoldToDelete=off, PLCVarF3DownBHoldName=F3DownBHold, PLCVarF3DownBHoldScope=Local, PLCVarF3DownBHoldPortType=Hidden, PLCVarF3DownBHoldPortIndex=59, PLCVarF3DownBHoldDataType=BOOL, PLCVarF3DownBHoldSize=1, PLCVarF3DownBHoldInitialValue=false, PLCVarF3DownBHoldToDelete=off, PLCVarF3PBHoldName=F3PBHold, PLCVarF3PBHoldScope=Local, PLCVarF3PBHoldPortType=Hidden, PLCVarF3PBHoldPortIndex=59, PLCVarF3PBHoldDataType=BOOL, PLCVarF3PBHoldSize=1, PLCVarF3PBHoldInitialValue=false, PLCVarF3PBHoldToDelete=off, PLCVarFloor_1Name=Floor_1, PLCVarFloor_1Scope=Local, PLCVarFloor_1PortType=Hidden, PLCVarFloor_1PortIndex=59, PLCVarFloor_1DataType=DINT, PLCVarFloor_1Size=1, PLCVarFloor_1InitialValue=1, PLCVarFloor_1ToDelete=off, PLCVarFloor_2Name=Floor_2, PLCVarFloor_2Scope=Local, PLCVarFloor_2PortType=Hidden, PLCVarFloor_2PortIndex=59, PLCVarFloor_2DataType=DINT, PLCVarFloor_2Size=1, PLCVarFloor_2InitialValue=2, PLCVarFloor_2ToDelete=off, PLCVarFloor_3Name=Floor_3, PLCVarFloor_3Scope=Local, PLCVarFloor_3PortType=Hidden, PLCVarFloor_3PortIndex=59, PLCVarFloor_3DataType=DINT, PLCVarFloor_3Size=1, PLCVarFloor_3InitialValue=3, PLCVarFloor_3ToDelete=off, PLCVarGOINGDNName=GOINGDN, PLCVarGOINGDNScope=Local, PLCVarGOINGDNPortType=Hidden, PLCVarGOINGDNPortIndex=59, PLCVarGOINGDNDataType=BOOL, PLCVarGOINGDNSize=1, PLCVarGOINGDNInitialValue=false, PLCVarGOINGDNToDelete=off, PLCVarGOINGUPName=GOINGUP, PLCVarGOINGUPScope=Local, PLCVarGOINGUPPortType=Hidden, PLCVarGOINGUPPortIndex=59, PLCVarGOINGUPDataType=BOOL, PLCVarGOINGUPSize=1, PLCVarGOINGUPInitialValue=false, PLCVarGOINGUPToDelete=off, PLCVarINCSPDName=INCSPD, PLCVarINCSPDScope=Local, PLCVarINCSPDPortType=Hidden, PLCVarINCSPDPortIndex=59, PLCVarINCSPDDataType=BOOL, PLCVarINCSPDSize=1, PLCVarINCSPDInitialValue=false, PLCVarINCSPDToDelete=off, PLCVarLSTDIRUPName=LSTDIRUP, PLCVarLSTDIRUPScope=Local, PLCVarLSTDIRUPPortType=Hidden, PLCVarLSTDIRUPPortIndex=59, PLCVarLSTDIRUPDataType=BOOL, PLCVarLSTDIRUPSize=1, PLCVarLSTDIRUPInitialValue=false, PLCVarLSTDIRUPToDelete=off, PLCVarMTRONName=MTRON, PLCVarMTRONScope=Local, PLCVarMTRONPortType=Hidden, PLCVarMTRONPortIndex=59, PLCVarMTRONDataType=BOOL, PLCVarMTRONSize=1, PLCVarMTRONInitialValue=false, PLCVarMTRONToDelete=off, PLCVarMemoryGoDownName=MemoryGoDown, PLCVarMemoryGoDownScope=Local, PLCVarMemoryGoDownPortType=Hidden, PLCVarMemoryGoDownPortIndex=59, PLCVarMemoryGoDownDataType=BOOL, PLCVarMemoryGoDownSize=1, PLCVarMemoryGoDownInitialValue=false, PLCVarMemoryGoDownToDelete=off, PLCVarMemoryGoUpName=MemoryGoUp, PLCVarMemoryGoUpScope=Local, PLCVarMemoryGoUpPortType=Hidden, PLCVarMemoryGoUpPortIndex=59, PLCVarMemoryGoUpDataType=BOOL, PLCVarMemoryGoUpSize=1, PLCVarMemoryGoUpInitialValue=false, PLCVarMemoryGoUpToDelete=off, PLCVarRMPDNName=RMPDN, PLCVarRMPDNScope=Local, PLCVarRMPDNPortType=Hidden, PLCVarRMPDNPortIndex=59, PLCVarRMPDNDataType=BOOL, PLCVarRMPDNSize=1, PLCVarRMPDNInitialValue=false, PLCVarRMPDNToDelete=off, PLCVarRMPDNKILName=RMPDNKIL, PLCVarRMPDNKILScope=Local, PLCVarRMPDNKILPortType=Hidden, PLCVarRMPDNKILPortIndex=59, PLCVarRMPDNKILDataType=BOOL, PLCVarRMPDNKILSize=1, PLCVarRMPDNKILInitialValue=false, PLCVarRMPDNKILToDelete=off, PLCVarRMPDNTRGName=RMPDNTRG, PLCVarRMPDNTRGScope=Local, PLCVarRMPDNTRGPortType=Hidden, PLCVarRMPDNTRGPortIndex=59, PLCVarRMPDNTRGDataType=BOOL, PLCVarRMPDNTRGSize=1, PLCVarRMPDNTRGInitialValue=false, PLCVarRMPDNTRGToDelete=off, PLCVarRMPUPName=RMPUP, PLCVarRMPUPScope=Local, PLCVarRMPUPPortType=Hidden, PLCVarRMPUPPortIndex=59, PLCVarRMPUPDataType=BOOL, PLCVarRMPUPSize=1, PLCVarRMPUPInitialValue=false, PLCVarRMPUPToDelete=off, PLCVarRMPUPKILName=RMPUPKIL, PLCVarRMPUPKILScope=Local, PLCVarRMPUPKILPortType=Hidden, PLCVarRMPUPKILPortIndex=59, PLCVarRMPUPKILDataType=BOOL, PLCVarRMPUPKILSize=1, PLCVarRMPUPKILInitialValue=false, PLCVarRMPUPKILToDelete=off, PLCVarRMPUPTRGName=RMPUPTRG, PLCVarRMPUPTRGScope=Local, PLCVarRMPUPTRGPortType=Hidden, PLCVarRMPUPTRGPortIndex=59, PLCVarRMPUPTRGDataType=BOOL, PLCVarRMPUPTRGSize=1, PLCVarRMPUPTRGInitialValue=false, PLCVarRMPUPTRGToDelete=off, PLCVarSENCHKName=SENCHK, PLCVarSENCHKScope=Local, PLCVarSENCHKPortType=Hidden, PLCVarSENCHKPortIndex=59, PLCVarSENCHKDataType=BOOL, PLCVarSENCHKSize=1, PLCVarSENCHKInitialValue=false, PLCVarSENCHKToDelete=off, PLCVarStartHoldName=StartHold, PLCVarStartHoldScope=Local, PLCVarStartHoldPortType=Hidden, PLCVarStartHoldPortIndex=59, PLCVarStartHoldDataType=BOOL, PLCVarStartHoldSize=1, PLCVarStartHoldInitialValue=false, PLCVarStartHoldToDelete=off, PLCVarTName=T, PLCVarTScope=Local, PLCVarTPortType=Hidden, PLCVarTPortIndex=59, PLCVarTDataType=Bus: TIMER, PLCVarTSize=1, PLCVarTInitialValue=TON_InitialValue, PLCVarTToDelete=off, PLCVarTempS1HName=TempS1H, PLCVarTempS1HScope=Local, PLCVarTempS1HPortType=Hidden, PLCVarTempS1HPortIndex=59, PLCVarTempS1HDataType=BOOL, PLCVarTempS1HSize=1, PLCVarTempS1HInitialValue=false, PLCVarTempS1HToDelete=off, PLCVarTempS1HDownName=TempS1HDown, PLCVarTempS1HDownScope=Local, PLCVarTempS1HDownPortType=Hidden, PLCVarTempS1HDownPortIndex=59, PLCVarTempS1HDownDataType=BOOL, PLCVarTempS1HDownSize=1, PLCVarTempS1HDownInitialValue=false, PLCVarTempS1HDownToDelete=off, PLCVarTempS1HUpName=TempS1HUp, PLCVarTempS1HUpScope=Local, PLCVarTempS1HUpPortType=Hidden, PLCVarTempS1HUpPortIndex=59, PLCVarTempS1HUpDataType=BOOL, PLCVarTempS1HUpSize=1, PLCVarTempS1HUpInitialValue=false, PLCVarTempS1HUpToDelete=off, PLCVarTempS1HupName=TempS1Hup, PLCVarTempS1HupScope=Local, PLCVarTempS1HupPortType=Hidden, PLCVarTempS1HupPortIndex=59, PLCVarTempS1HupDataType=BOOL, PLCVarTempS1HupSize=1, PLCVarTempS1HupInitialValue=false, PLCVarTempS1HupToDelete=off, PLCVarTempS2HName=TempS2H, PLCVarTempS2HScope=Local, PLCVarTempS2HPortType=Hidden, PLCVarTempS2HPortIndex=59, PLCVarTempS2HDataType=BOOL, PLCVarTempS2HSize=1, PLCVarTempS2HInitialValue=false, PLCVarTempS2HToDelete=off, PLCVarTempS2HDownName=TempS2HDown, PLCVarTempS2HDownScope=Local, PLCVarTempS2HDownPortType=Hidden, PLCVarTempS2HDownPortIndex=59, PLCVarTempS2HDownDataType=BOOL, PLCVarTempS2HDownSize=1, PLCVarTempS2HDownInitialValue=false, PLCVarTempS2HDownToDelete=off, PLCVarTempS2HUpName=TempS2HUp, PLCVarTempS2HUpScope=Local, PLCVarTempS2HUpPortType=Hidden, PLCVarTempS2HUpPortIndex=59, PLCVarTempS2HUpDataType=BOOL, PLCVarTempS2HUpSize=1, PLCVarTempS2HUpInitialValue=false, PLCVarTempS2HUpToDelete=off, PLCVarTempS2LName=TempS2L, PLCVarTempS2LScope=Local, PLCVarTempS2LPortType=Hidden, PLCVarTempS2LPortIndex=59, PLCVarTempS2LDataType=BOOL, PLCVarTempS2LSize=1, PLCVarTempS2LInitialValue=false, PLCVarTempS2LToDelete=off, PLCVarTempS2LDownName=TempS2LDown, PLCVarTempS2LDownScope=Local, PLCVarTempS2LDownPortType=Hidden, PLCVarTempS2LDownPortIndex=59, PLCVarTempS2LDownDataType=BOOL, PLCVarTempS2LDownSize=1, PLCVarTempS2LDownInitialValue=false, PLCVarTempS2LDownToDelete=off, PLCVarTempS2LUpName=TempS2LUp, PLCVarTempS2LUpScope=Local, PLCVarTempS2LUpPortType=Hidden, PLCVarTempS2LUpPortIndex=59, PLCVarTempS2LUpDataType=BOOL, PLCVarTempS2LUpSize=1, PLCVarTempS2LUpInitialValue=false, PLCVarTempS2LUpToDelete=off, PLCVarTempS3LName=TempS3L, PLCVarTempS3LScope=Local, PLCVarTempS3LPortType=Hidden, PLCVarTempS3LPortIndex=59, PLCVarTempS3LDataType=BOOL, PLCVarTempS3LSize=1, PLCVarTempS3LInitialValue=false, PLCVarTempS3LToDelete=off, PLCVarTempS3LDownName=TempS3LDown, PLCVarTempS3LDownScope=Local, PLCVarTempS3LDownPortType=Hidden, PLCVarTempS3LDownPortIndex=59, PLCVarTempS3LDownDataType=BOOL, PLCVarTempS3LDownSize=1, PLCVarTempS3LDownInitialValue=false, PLCVarTempS3LDownToDelete=off, PLCVarTempS3LUpName=TempS3LUp, PLCVarTempS3LUpScope=Local, PLCVarTempS3LUpPortType=Hidden, PLCVarTempS3LUpPortIndex=59, PLCVarTempS3LUpDataType=BOOL, PLCVarTempS3LUpSize=1, PLCVarTempS3LUpInitialValue=false, PLCVarTempS3LUpToDelete=off, PLCVarVARVELName=VARVEL, PLCVarVARVELScope=Local, PLCVarVARVELPortType=Hidden, PLCVarVARVELPortIndex=59, PLCVarVARVELDataType=single, PLCVarVARVELSize=1, PLCVarVARVELInitialValue=0.0, PLCVarVARVELToDelete=off, PLCVarF1PBName=F1PB, PLCVarF1PBScope=External, PLCVarF1PBPortType=Hidden, PLCVarF1PBPortIndex=59, PLCVarF1PBDataType=DINT, PLCVarF1PBSize=-1, PLCVarF1PBInitialValue=0, PLCVarF1PBToDelete=off, PLCVarF1UpBName=F1UpB, PLCVarF1UpBScope=External, PLCVarF1UpBPortType=Hidden, PLCVarF1UpBPortIndex=59, PLCVarF1UpBDataType=DINT, PLCVarF1UpBSize=-1, PLCVarF1UpBInitialValue=0, PLCVarF1UpBToDelete=off, PLCVarF2DownBName=F2DownB, PLCVarF2DownBScope=External, PLCVarF2DownBPortType=Hidden, PLCVarF2DownBPortIndex=59, PLCVarF2DownBDataType=DINT, PLCVarF2DownBSize=-1, PLCVarF2DownBInitialValue=0, PLCVarF2DownBToDelete=off, PLCVarF2PBName=F2PB, PLCVarF2PBScope=External, PLCVarF2PBPortType=Hidden, PLCVarF2PBPortIndex=59, PLCVarF2PBDataType=DINT, PLCVarF2PBSize=-1, PLCVarF2PBInitialValue=0, PLCVarF2PBToDelete=off, PLCVarF2UpBName=F2UpB, PLCVarF2UpBScope=External, PLCVarF2UpBPortType=Hidden, PLCVarF2UpBPortIndex=59, PLCVarF2UpBDataType=DINT, PLCVarF2UpBSize=-1, PLCVarF2UpBInitialValue=0, PLCVarF2UpBToDelete=off, PLCVarF3DownBName=F3DownB, PLCVarF3DownBScope=External, PLCVarF3DownBPortType=Hidden, PLCVarF3DownBPortIndex=59, PLCVarF3DownBDataType=DINT, PLCVarF3DownBSize=-1, PLCVarF3DownBInitialValue=0, PLCVarF3DownBToDelete=off, PLCVarF3PBName=F3PB, PLCVarF3PBScope=External, PLCVarF3PBPortType=Hidden, PLCVarF3PBPortIndex=59, PLCVarF3PBDataType=DINT, PLCVarF3PBSize=-1, PLCVarF3PBInitialValue=0, PLCVarF3PBToDelete=off, PLCVarFLOOROUTName=FLOOROUT, PLCVarFLOOROUTScope=External, PLCVarFLOOROUTPortType=Hidden, PLCVarFLOOROUTPortIndex=59, PLCVarFLOOROUTDataType=DINT, PLCVarFLOOROUTSize=-1, PLCVarFLOOROUTInitialValue=0, PLCVarFLOOROUTToDelete=off, PLCVarS1HName=S1H, PLCVarS1HScope=External, PLCVarS1HPortType=Hidden, PLCVarS1HPortIndex=59, PLCVarS1HDataType=DINT, PLCVarS1HSize=-1, PLCVarS1HInitialValue=0, PLCVarS1HToDelete=off, PLCVarS2HName=S2H, PLCVarS2HScope=External, PLCVarS2HPortType=Hidden, PLCVarS2HPortIndex=59, PLCVarS2HDataType=DINT, PLCVarS2HSize=-1, PLCVarS2HInitialValue=0, PLCVarS2HToDelete=off, PLCVarS2LName=S2L, PLCVarS2LScope=External, PLCVarS2LPortType=Hidden, PLCVarS2LPortIndex=59, PLCVarS2LDataType=DINT, PLCVarS2LSize=-1, PLCVarS2LInitialValue=0, PLCVarS2LToDelete=off, PLCVarS3LName=S3L, PLCVarS3LScope=External, PLCVarS3LPortType=Hidden, PLCVarS3LPortIndex=59, PLCVarS3LDataType=DINT, PLCVarS3LSize=-1, PLCVarS3LInitialValue=0, PLCVarS3LToDelete=off, PLCVarStartName=Start, PLCVarStartScope=External, PLCVarStartPortType=Hidden, PLCVarStartPortIndex=59, PLCVarStartDataType=DINT, PLCVarStartSize=-1, PLCVarStartInitialValue=0, PLCVarStartToDelete=off, PLCVarStopName=Stop, PLCVarStopScope=External, PLCVarStopPortType=Hidden, PLCVarStopPortIndex=59, PLCVarStopDataType=DINT, PLCVarStopSize=-1, PLCVarStopInitialValue=0, PLCVarStopToDelete=off, PLCVarVELOUTName=VELOUT, PLCVarVELOUTScope=External, PLCVarVELOUTPortType=Hidden, PLCVarVELOUTPortIndex=59, PLCVarVELOUTDataType=DINT, PLCVarVELOUTSize=-1, PLCVarVELOUTInitialValue=0, PLCVarVELOUTToDelete=off}
      mask init:
      | slplc.callbacks.initPOUVarSS(gcb);
      settings: OpenFcn=slplc.callbacks.openProgramVariableSS(gcb);
      mask Help: web([docroot '/plccoder/ref/programvariables' '.html']);
      mask TypeOptions PLCVarAtFloor1Scope: Local | External
      mask Callback PLCVarAtFloor1Scope: slplc.callbacks.updatePOUVarSS(gcb);
      mask TypeOptions PLCVarAtFloor1PortType: Hidden | Inport | Outport
      mask Callback PLCVarAtFloor1PortType: slplc.callbacks.updatePOUVarSS(gcb);
      mask TypeOptions PLCVarAtFloor1PortIndex: 1 | 2 | 3 | 4 | 5 | 6 | 7 | 8 | 9 | 10 | 11 | 12 | 13 | 14 | 15 | 16 | 17 | 18 | 19 | 20 | 21 | 22 | 23 | 24 | 25 | 26 | 27 | 28 | 29 | 30 | 31 | 32 | 33 | 34 | 35 | 36 | 37 | 38 | 39 | 40 | 41 | 42 | 43 | 44 | 45 | 46 | 47 | 48 | 49 | 50 | 51 | 52 | 53 | 54 | 55 | 56 | 57 | 58 | 59
      mask TypeOptions PLCVarAtFloor2Scope: Local | External
      mask Callback PLCVarAtFloor2Scope: slplc.callbacks.updatePOUVarSS(gcb);
      mask TypeOptions PLCVarAtFloor2PortType: Hidden | Inport | Outport
      mask Callback PLCVarAtFloor2PortType: slplc.callbacks.updatePOUVarSS(gcb);
      mask TypeOptions PLCVarAtFloor2PortIndex: 1 | 2 | 3 | 4 | 5 | 6 | 7 | 8 | 9 | 10 | 11 | 12 | 13 | 14 | 15 | 16 | 17 | 18 | 19 | 20 | 21 | 22 | 23 | 24 | 25 | 26 | 27 | 28 | 29 | 30 | 31 | 32 | 33 | 34 | 35 | 36 | 37 | 38 | 39 | 40 | 41 | 42 | 43 | 44 | 45 | 46 | 47 | 48 | 49 | 50 | 51 | 52 | 53 | 54 | 55 | 56 | 57 | 58 | 59
      mask TypeOptions PLCVarAtFloor3Scope: Local | External
      mask Callback PLCVarAtFloor3Scope: slplc.callbacks.updatePOUVarSS(gcb);
      mask TypeOptions PLCVarAtFloor3PortType: Hidden | Inport | Outport
      mask Callback PLCVarAtFloor3PortType: slplc.callbacks.updatePOUVarSS(gcb);
      mask TypeOptions PLCVarAtFloor3PortIndex: 1 | 2 | 3 | 4 | 5 | 6 | 7 | 8 | 9 | 10 | 11 | 12 | 13 | 14 | 15 | 16 | 17 | 18 | 19 | 20 | 21 | 22 | 23 | 24 | 25 | 26 | 27 | 28 | 29 | 30 | 31 | 32 | 33 | 34 | 35 | 36 | 37 | 38 | 39 | 40 | 41 | 42 | 43 | 44 | 45 | 46 | 47 | 48 | 49 | 50 | 51 | 52 | 53 | 54 | 55 | 56 | 57 | 58 | 59
      mask TypeOptions PLCVarCurrent_floorScope: Local | External
      mask Callback PLCVarCurrent_floorScope: slplc.callbacks.updatePOUVarSS(gcb);
      mask TypeOptions PLCVarCurrent_floorPortType: Hidden | Inport | Outport
      mask Callback PLCVarCurrent_floorPortType: slplc.callbacks.updatePOUVarSS(gcb);
      mask TypeOptions PLCVarCurrent_floorPortIndex: 1 | 2 | 3 | 4 | 5 | 6 | 7 | 8 | 9 | 10 | 11 | 12 | 13 | 14 | 15 | 16 | 17 | 18 | 19 | 20 | 21 | 22 | 23 | 24 | 25 | 26 | 27 | 28 | 29 | 30 | 31 | 32 | 33 | 34 | 35 | 36 | 37 | 38 | 39 | 40 | 41 | 42 | 43 | 44 | 45 | 46 | 47 | 48 | 49 | 50 | 51 | 52 | 53 | 54 | 55 | 56 | 57 | 58 | 59
      mask TypeOptions PLCVarDECSPDScope: Local | External
      mask Callback PLCVarDECSPDScope: slplc.callbacks.updatePOUVarSS(gcb);
      mask TypeOptions PLCVarDECSPDPortType: Hidden | Inport | Outport
      mask Callback PLCVarDECSPDPortType: slplc.callbacks.updatePOUVarSS(gcb);
      mask TypeOptions PLCVarDECSPDPortIndex: 1 | 2 | 3 | 4 | 5 | 6 | 7 | 8 | 9 | 10 | 11 | 12 | 13 | 14 | 15 | 16 | 17 | 18 | 19 | 20 | 21 | 22 | 23 | 24 | 25 | 26 | 27 | 28 | 29 | 30 | 31 | 32 | 33 | 34 | 35 | 36 | 37 | 38 | 39 | 40 | 41 | 42 | 43 | 44 | 45 | 46 | 47 | 48 | 49 | 50 | 51 | 52 | 53 | 54 | 55 | 56 | 57 | 58 | 59
      mask TypeOptions PLCVarF1PBHoldScope: Local | External
      mask Callback PLCVarF1PBHoldScope: slplc.callbacks.updatePOUVarSS(gcb);
      mask TypeOptions PLCVarF1PBHoldPortType: Hidden | Inport | Outport
      mask Callback PLCVarF1PBHoldPortType: slplc.callbacks.updatePOUVarSS(gcb);
      mask TypeOptions PLCVarF1PBHoldPortIndex: 1 | 2 | 3 | 4 | 5 | 6 | 7 | 8 | 9 | 10 | 11 | 12 | 13 | 14 | 15 | 16 | 17 | 18 | 19 | 20 | 21 | 22 | 23 | 24 | 25 | 26 | 27 | 28 | 29 | 30 | 31 | 32 | 33 | 34 | 35 | 36 | 37 | 38 | 39 | 40 | 41 | 42 | 43 | 44 | 45 | 46 | 47 | 48 | 49 | 50 | 51 | 52 | 53 | 54 | 55 | 56 | 57 | 58 | 59
      mask TypeOptions PLCVarF1UpBHoldScope: Local | External
      mask Callback PLCVarF1UpBHoldScope: slplc.callbacks.updatePOUVarSS(gcb);
      mask TypeOptions PLCVarF1UpBHoldPortType: Hidden | Inport | Outport
      mask Callback PLCVarF1UpBHoldPortType: slplc.callbacks.updatePOUVarSS(gcb);
      mask TypeOptions PLCVarF1UpBHoldPortIndex: 1 | 2 | 3 | 4 | 5 | 6 | 7 | 8 | 9 | 10 | 11 | 12 | 13 | 14 | 15 | 16 | 17 | 18 | 19 | 20 | 21 | 22 | 23 | 24 | 25 | 26 | 27 | 28 | 29 | 30 | 31 | 32 | 33 | 34 | 35 | 36 | 37 | 38 | 39 | 40 | 41 | 42 | 43 | 44 | 45 | 46 | 47 | 48 | 49 | 50 | 51 | 52 | 53 | 54 | 55 | 56 | 57 | 58 | 59
      mask TypeOptions PLCVarF2PBHoldScope: Local | External
      mask Callback PLCVarF2PBHoldScope: slplc.callbacks.updatePOUVarSS(gcb);
      mask TypeOptions PLCVarF2PBHoldPortType: Hidden | Inport | Outport
      mask Callback PLCVarF2PBHoldPortType: slplc.callbacks.updatePOUVarSS(gcb);
      mask TypeOptions PLCVarF2PBHoldPortIndex: 1 | 2 | 3 | 4 | 5 | 6 | 7 | 8 | 9 | 10 | 11 | 12 | 13 | 14 | 15 | 16 | 17 | 18 | 19 | 20 | 21 | 22 | 23 | 24 | 25 | 26 | 27 | 28 | 29 | 30 | 31 | 32 | 33 | 34 | 35 | 36 | 37 | 38 | 39 | 40 | 41 | 42 | 43 | 44 | 45 | 46 | 47 | 48 | 49 | 50 | 51 | 52 | 53 | 54 | 55 | 56 | 57 | 58 | 59
      mask TypeOptions PLCVarF2UpDownBHoldScope: Local | External
      mask Callback PLCVarF2UpDownBHoldScope: slplc.callbacks.updatePOUVarSS(gcb);
      mask TypeOptions PLCVarF2UpDownBHoldPortType: Hidden | Inport | Outport
      mask Callback PLCVarF2UpDownBHoldPortType: slplc.callbacks.updatePOUVarSS(gcb);
      mask TypeOptions PLCVarF2UpDownBHoldPortIndex: 1 | 2 | 3 | 4 | 5 | 6 | 7 | 8 | 9 | 10 | 11 | 12 | 13 | 14 | 15 | 16 | 17 | 18 | 19 | 20 | 21 | 22 | 23 | 24 | 25 | 26 | 27 | 28 | 29 | 30 | 31 | 32 | 33 | 34 | 35 | 36 | 37 | 38 | 39 | 40 | 41 | 42 | 43 | 44 | 45 | 46 | 47 | 48 | 49 | 50 | 51 | 52 | 53 | 54 | 55 | 56 | 57 | 58 | 59
      mask TypeOptions PLCVarF3DownBHoldScope: Local | External
      mask Callback PLCVarF3DownBHoldScope: slplc.callbacks.updatePOUVarSS(gcb);
      mask TypeOptions PLCVarF3DownBHoldPortType: Hidden | Inport | Outport
      mask Callback PLCVarF3DownBHoldPortType: slplc.callbacks.updatePOUVarSS(gcb);
      mask TypeOptions PLCVarF3DownBHoldPortIndex: 1 | 2 | 3 | 4 | 5 | 6 | 7 | 8 | 9 | 10 | 11 | 12 | 13 | 14 | 15 | 16 | 17 | 18 | 19 | 20 | 21 | 22 | 23 | 24 | 25 | 26 | 27 | 28 | 29 | 30 | 31 | 32 | 33 | 34 | 35 | 36 | 37 | 38 | 39 | 40 | 41 | 42 | 43 | 44 | 45 | 46 | 47 | 48 | 49 | 50 | 51 | 52 | 53 | 54 | 55 | 56 | 57 | 58 | 59
      mask TypeOptions PLCVarF3PBHoldScope: Local | External
      mask Callback PLCVarF3PBHoldScope: slplc.callbacks.updatePOUVarSS(gcb);
      mask TypeOptions PLCVarF3PBHoldPortType: Hidden | Inport | Outport
      mask Callback PLCVarF3PBHoldPortType: slplc.callbacks.updatePOUVarSS(gcb);
      mask TypeOptions PLCVarF3PBHoldPortIndex: 1 | 2 | 3 | 4 | 5 | 6 | 7 | 8 | 9 | 10 | 11 | 12 | 13 | 14 | 15 | 16 | 17 | 18 | 19 | 20 | 21 | 22 | 23 | 24 | 25 | 26 | 27 | 28 | 29 | 30 | 31 | 32 | 33 | 34 | 35 | 36 | 37 | 38 | 39 | 40 | 41 | 42 | 43 | 44 | 45 | 46 | 47 | 48 | 49 | 50 | 51 | 52 | 53 | 54 | 55 | 56 | 57 | 58 | 59
      mask TypeOptions PLCVarFloor_1Scope: Local | External
      mask Callback PLCVarFloor_1Scope: slplc.callbacks.updatePOUVarSS(gcb);
      mask TypeOptions PLCVarFloor_1PortType: Hidden | Inport | Outport
      mask Callback PLCVarFloor_1PortType: slplc.callbacks.updatePOUVarSS(gcb);
      mask TypeOptions PLCVarFloor_1PortIndex: 1 | 2 | 3 | 4 | 5 | 6 | 7 | 8 | 9 | 10 | 11 | 12 | 13 | 14 | 15 | 16 | 17 | 18 | 19 | 20 | 21 | 22 | 23 | 24 | 25 | 26 | 27 | 28 | 29 | 30 | 31 | 32 | 33 | 34 | 35 | 36 | 37 | 38 | 39 | 40 | 41 | 42 | 43 | 44 | 45 | 46 | 47 | 48 | 49 | 50 | 51 | 52 | 53 | 54 | 55 | 56 | 57 | 58 | 59
      mask TypeOptions PLCVarFloor_2Scope: Local | External
      mask Callback PLCVarFloor_2Scope: slplc.callbacks.updatePOUVarSS(gcb);
      mask TypeOptions PLCVarFloor_2PortType: Hidden | Inport | Outport
      mask Callback PLCVarFloor_2PortType: slplc.callbacks.updatePOUVarSS(gcb);
      mask TypeOptions PLCVarFloor_2PortIndex: 1 | 2 | 3 | 4 | 5 | 6 | 7 | 8 | 9 | 10 | 11 | 12 | 13 | 14 | 15 | 16 | 17 | 18 | 19 | 20 | 21 | 22 | 23 | 24 | 25 | 26 | 27 | 28 | 29 | 30 | 31 | 32 | 33 | 34 | 35 | 36 | 37 | 38 | 39 | 40 | 41 | 42 | 43 | 44 | 45 | 46 | 47 | 48 | 49 | 50 | 51 | 52 | 53 | 54 | 55 | 56 | 57 | 58 | 59
      mask TypeOptions PLCVarFloor_3Scope: Local | External
      mask Callback PLCVarFloor_3Scope: slplc.callbacks.updatePOUVarSS(gcb);
      mask TypeOptions PLCVarFloor_3PortType: Hidden | Inport | Outport
      mask Callback PLCVarFloor_3PortType: slplc.callbacks.updatePOUVarSS(gcb);
      mask TypeOptions PLCVarFloor_3PortIndex: 1 | 2 | 3 | 4 | 5 | 6 | 7 | 8 | 9 | 10 | 11 | 12 | 13 | 14 | 15 | 16 | 17 | 18 | 19 | 20 | 21 | 22 | 23 | 24 | 25 | 26 | 27 | 28 | 29 | 30 | 31 | 32 | 33 | 34 | 35 | 36 | 37 | 38 | 39 | 40 | 41 | 42 | 43 | 44 | 45 | 46 | 47 | 48 | 49 | 50 | 51 | 52 | 53 | 54 | 55 | 56 | 57 | 58 | 59
      mask TypeOptions PLCVarGOINGDNScope: Local | External
      mask Callback PLCVarGOINGDNScope: slplc.callbacks.updatePOUVarSS(gcb);
      mask TypeOptions PLCVarGOINGDNPortType: Hidden | Inport | Outport
      mask Callback PLCVarGOINGDNPortType: slplc.callbacks.updatePOUVarSS(gcb);
      mask TypeOptions PLCVarGOINGDNPortIndex: 1 | 2 | 3 | 4 | 5 | 6 | 7 | 8 | 9 | 10 | 11 | 12 | 13 | 14 | 15 | 16 | 17 | 18 | 19 | 20 | 21 | 22 | 23 | 24 | 25 | 26 | 27 | 28 | 29 | 30 | 31 | 32 | 33 | 34 | 35 | 36 | 37 | 38 | 39 | 40 | 41 | 42 | 43 | 44 | 45 | 46 | 47 | 48 | 49 | 50 | 51 | 52 | 53 | 54 | 55 | 56 | 57 | 58 | 59
      mask TypeOptions PLCVarGOINGUPScope: Local | External
      mask Callback PLCVarGOINGUPScope: slplc.callbacks.updatePOUVarSS(gcb);
      mask TypeOptions PLCVarGOINGUPPortType: Hidden | Inport | Outport
      mask Callback PLCVarGOINGUPPortType: slplc.callbacks.updatePOUVarSS(gcb);
      mask TypeOptions PLCVarGOINGUPPortIndex: 1 | 2 | 3 | 4 | 5 | 6 | 7 | 8 | 9 | 10 | 11 | 12 | 13 | 14 | 15 | 16 | 17 | 18 | 19 | 20 | 21 | 22 | 23 | 24 | 25 | 26 | 27 | 28 | 29 | 30 | 31 | 32 | 33 | 34 | 35 | 36 | 37 | 38 | 39 | 40 | 41 | 42 | 43 | 44 | 45 | 46 | 47 | 48 | 49 | 50 | 51 | 52 | 53 | 54 | 55 | 56 | 57 | 58 | 59
      mask TypeOptions PLCVarINCSPDScope: Local | External
      mask Callback PLCVarINCSPDScope: slplc.callbacks.updatePOUVarSS(gcb);
      mask TypeOptions PLCVarINCSPDPortType: Hidden | Inport | Outport
      mask Callback PLCVarINCSPDPortType: slplc.callbacks.updatePOUVarSS(gcb);
      mask TypeOptions PLCVarINCSPDPortIndex: 1 | 2 | 3 | 4 | 5 | 6 | 7 | 8 | 9 | 10 | 11 | 12 | 13 | 14 | 15 | 16 | 17 | 18 | 19 | 20 | 21 | 22 | 23 | 24 | 25 | 26 | 27 | 28 | 29 | 30 | 31 | 32 | 33 | 34 | 35 | 36 | 37 | 38 | 39 | 40 | 41 | 42 | 43 | 44 | 45 | 46 | 47 | 48 | 49 | 50 | 51 | 52 | 53 | 54 | 55 | 56 | 57 | 58 | 59
      mask TypeOptions PLCVarLSTDIRUPScope: Local | External
      mask Callback PLCVarLSTDIRUPScope: slplc.callbacks.updatePOUVarSS(gcb);
      mask TypeOptions PLCVarLSTDIRUPPortType: Hidden | Inport | Outport
      mask Callback PLCVarLSTDIRUPPortType: slplc.callbacks.updatePOUVarSS(gcb);
      mask TypeOptions PLCVarLSTDIRUPPortIndex: 1 | 2 | 3 | 4 | 5 | 6 | 7 | 8 | 9 | 10 | 11 | 12 | 13 | 14 | 15 | 16 | 17 | 18 | 19 | 20 | 21 | 22 | 23 | 24 | 25 | 26 | 27 | 28 | 29 | 30 | 31 | 32 | 33 | 34 | 35 | 36 | 37 | 38 | 39 | 40 | 41 | 42 | 43 | 44 | 45 | 46 | 47 | 48 | 49 | 50 | 51 | 52 | 53 | 54 | 55 | 56 | 57 | 58 | 59
      mask TypeOptions PLCVarMTRONScope: Local | External
      mask Callback PLCVarMTRONScope: slplc.callbacks.updatePOUVarSS(gcb);
      mask TypeOptions PLCVarMTRONPortType: Hidden | Inport | Outport
      mask Callback PLCVarMTRONPortType: slplc.callbacks.updatePOUVarSS(gcb);
      mask TypeOptions PLCVarMTRONPortIndex: 1 | 2 | 3 | 4 | 5 | 6 | 7 | 8 | 9 | 10 | 11 | 12 | 13 | 14 | 15 | 16 | 17 | 18 | 19 | 20 | 21 | 22 | 23 | 24 | 25 | 26 | 27 | 28 | 29 | 30 | 31 | 32 | 33 | 34 | 35 | 36 | 37 | 38 | 39 | 40 | 41 | 42 | 43 | 44 | 45 | 46 | 47 | 48 | 49 | 50 | 51 | 52 | 53 | 54 | 55 | 56 | 57 | 58 | 59
      mask TypeOptions PLCVarMemoryGoDownScope: Local | External
      mask Callback PLCVarMemoryGoDownScope: slplc.callbacks.updatePOUVarSS(gcb);
      mask TypeOptions PLCVarMemoryGoDownPortType: Hidden | Inport | Outport
      mask Callback PLCVarMemoryGoDownPortType: slplc.callbacks.updatePOUVarSS(gcb);
      mask TypeOptions PLCVarMemoryGoDownPortIndex: 1 | 2 | 3 | 4 | 5 | 6 | 7 | 8 | 9 | 10 | 11 | 12 | 13 | 14 | 15 | 16 | 17 | 18 | 19 | 20 | 21 | 22 | 23 | 24 | 25 | 26 | 27 | 28 | 29 | 30 | 31 | 32 | 33 | 34 | 35 | 36 | 37 | 38 | 39 | 40 | 41 | 42 | 43 | 44 | 45 | 46 | 47 | 48 | 49 | 50 | 51 | 52 | 53 | 54 | 55 | 56 | 57 | 58 | 59
      mask TypeOptions PLCVarMemoryGoUpScope: Local | External
      mask Callback PLCVarMemoryGoUpScope: slplc.callbacks.updatePOUVarSS(gcb);
      mask TypeOptions PLCVarMemoryGoUpPortType: Hidden | Inport | Outport
      mask Callback PLCVarMemoryGoUpPortType: slplc.callbacks.updatePOUVarSS(gcb);
      mask TypeOptions PLCVarMemoryGoUpPortIndex: 1 | 2 | 3 | 4 | 5 | 6 | 7 | 8 | 9 | 10 | 11 | 12 | 13 | 14 | 15 | 16 | 17 | 18 | 19 | 20 | 21 | 22 | 23 | 24 | 25 | 26 | 27 | 28 | 29 | 30 | 31 | 32 | 33 | 34 | 35 | 36 | 37 | 38 | 39 | 40 | 41 | 42 | 43 | 44 | 45 | 46 | 47 | 48 | 49 | 50 | 51 | 52 | 53 | 54 | 55 | 56 | 57 | 58 | 59
      mask TypeOptions PLCVarRMPDNScope: Local | External
      mask Callback PLCVarRMPDNScope: slplc.callbacks.updatePOUVarSS(gcb);
      mask TypeOptions PLCVarRMPDNPortType: Hidden | Inport | Outport
      mask Callback PLCVarRMPDNPortType: slplc.callbacks.updatePOUVarSS(gcb);
      mask TypeOptions PLCVarRMPDNPortIndex: 1 | 2 | 3 | 4 | 5 | 6 | 7 | 8 | 9 | 10 | 11 | 12 | 13 | 14 | 15 | 16 | 17 | 18 | 19 | 20 | 21 | 22 | 23 | 24 | 25 | 26 | 27 | 28 | 29 | 30 | 31 | 32 | 33 | 34 | 35 | 36 | 37 | 38 | 39 | 40 | 41 | 42 | 43 | 44 | 45 | 46 | 47 | 48 | 49 | 50 | 51 | 52 | 53 | 54 | 55 | 56 | 57 | 58 | 59
      mask TypeOptions PLCVarRMPDNKILScope: Local | External
      mask Callback PLCVarRMPDNKILScope: slplc.callbacks.updatePOUVarSS(gcb);
      mask TypeOptions PLCVarRMPDNKILPortType: Hidden | Inport | Outport
      mask Callback PLCVarRMPDNKILPortType: slplc.callbacks.updatePOUVarSS(gcb);
      mask TypeOptions PLCVarRMPDNKILPortIndex: 1 | 2 | 3 | 4 | 5 | 6 | 7 | 8 | 9 | 10 | 11 | 12 | 13 | 14 | 15 | 16 | 17 | 18 | 19 | 20 | 21 | 22 | 23 | 24 | 25 | 26 | 27 | 28 | 29 | 30 | 31 | 32 | 33 | 34 | 35 | 36 | 37 | 38 | 39 | 40 | 41 | 42 | 43 | 44 | 45 | 46 | 47 | 48 | 49 | 50 | 51 | 52 | 53 | 54 | 55 | 56 | 57 | 58 | 59
      mask TypeOptions PLCVarRMPDNTRGScope: Local | External
      mask Callback PLCVarRMPDNTRGScope: slplc.callbacks.updatePOUVarSS(gcb);
      mask TypeOptions PLCVarRMPDNTRGPortType: Hidden | Inport | Outport
      mask Callback PLCVarRMPDNTRGPortType: slplc.callbacks.updatePOUVarSS(gcb);
      mask TypeOptions PLCVarRMPDNTRGPortIndex: 1 | 2 | 3 | 4 | 5 | 6 | 7 | 8 | 9 | 10 | 11 | 12 | 13 | 14 | 15 | 16 | 17 | 18 | 19 | 20 | 21 | 22 | 23 | 24 | 25 | 26 | 27 | 28 | 29 | 30 | 31 | 32 | 33 | 34 | 35 | 36 | 37 | 38 | 39 | 40 | 41 | 42 | 43 | 44 | 45 | 46 | 47 | 48 | 49 | 50 | 51 | 52 | 53 | 54 | 55 | 56 | 57 | 58 | 59
      mask TypeOptions PLCVarRMPUPScope: Local | External
      mask Callback PLCVarRMPUPScope: slplc.callbacks.updatePOUVarSS(gcb);
      mask TypeOptions PLCVarRMPUPPortType: Hidden | Inport | Outport
      mask Callback PLCVarRMPUPPortType: slplc.callbacks.updatePOUVarSS(gcb);
      mask TypeOptions PLCVarRMPUPPortIndex: 1 | 2 | 3 | 4 | 5 | 6 | 7 | 8 | 9 | 10 | 11 | 12 | 13 | 14 | 15 | 16 | 17 | 18 | 19 | 20 | 21 | 22 | 23 | 24 | 25 | 26 | 27 | 28 | 29 | 30 | 31 | 32 | 33 | 34 | 35 | 36 | 37 | 38 | 39 | 40 | 41 | 42 | 43 | 44 | 45 | 46 | 47 | 48 | 49 | 50 | 51 | 52 | 53 | 54 | 55 | 56 | 57 | 58 | 59
      mask TypeOptions PLCVarRMPUPKILScope: Local | External
      mask Callback PLCVarRMPUPKILScope: slplc.callbacks.updatePOUVarSS(gcb);
      mask TypeOptions PLCVarRMPUPKILPortType: Hidden | Inport | Outport
      mask Callback PLCVarRMPUPKILPortType: slplc.callbacks.updatePOUVarSS(gcb);
      mask TypeOptions PLCVarRMPUPKILPortIndex: 1 | 2 | 3 | 4 | 5 | 6 | 7 | 8 | 9 | 10 | 11 | 12 | 13 | 14 | 15 | 16 | 17 | 18 | 19 | 20 | 21 | 22 | 23 | 24 | 25 | 26 | 27 | 28 | 29 | 30 | 31 | 32 | 33 | 34 | 35 | 36 | 37 | 38 | 39 | 40 | 41 | 42 | 43 | 44 | 45 | 46 | 47 | 48 | 49 | 50 | 51 | 52 | 53 | 54 | 55 | 56 | 57 | 58 | 59
      mask TypeOptions PLCVarRMPUPTRGScope: Local | External
      mask Callback PLCVarRMPUPTRGScope: slplc.callbacks.updatePOUVarSS(gcb);
      mask TypeOptions PLCVarRMPUPTRGPortType: Hidden | Inport | Outport
      mask Callback PLCVarRMPUPTRGPortType: slplc.callbacks.updatePOUVarSS(gcb);
      mask TypeOptions PLCVarRMPUPTRGPortIndex: 1 | 2 | 3 | 4 | 5 | 6 | 7 | 8 | 9 | 10 | 11 | 12 | 13 | 14 | 15 | 16 | 17 | 18 | 19 | 20 | 21 | 22 | 23 | 24 | 25 | 26 | 27 | 28 | 29 | 30 | 31 | 32 | 33 | 34 | 35 | 36 | 37 | 38 | 39 | 40 | 41 | 42 | 43 | 44 | 45 | 46 | 47 | 48 | 49 | 50 | 51 | 52 | 53 | 54 | 55 | 56 | 57 | 58 | 59
      mask TypeOptions PLCVarSENCHKScope: Local | External
      mask Callback PLCVarSENCHKScope: slplc.callbacks.updatePOUVarSS(gcb);
      mask TypeOptions PLCVarSENCHKPortType: Hidden | Inport | Outport
      mask Callback PLCVarSENCHKPortType: slplc.callbacks.updatePOUVarSS(gcb);
      mask TypeOptions PLCVarSENCHKPortIndex: 1 | 2 | 3 | 4 | 5 | 6 | 7 | 8 | 9 | 10 | 11 | 12 | 13 | 14 | 15 | 16 | 17 | 18 | 19 | 20 | 21 | 22 | 23 | 24 | 25 | 26 | 27 | 28 | 29 | 30 | 31 | 32 | 33 | 34 | 35 | 36 | 37 | 38 | 39 | 40 | 41 | 42 | 43 | 44 | 45 | 46 | 47 | 48 | 49 | 50 | 51 | 52 | 53 | 54 | 55 | 56 | 57 | 58 | 59
      mask TypeOptions PLCVarStartHoldScope: Local | External
      mask Callback PLCVarStartHoldScope: slplc.callbacks.updatePOUVarSS(gcb);
      mask TypeOptions PLCVarStartHoldPortType: Hidden | Inport | Outport
      mask Callback PLCVarStartHoldPortType: slplc.callbacks.updatePOUVarSS(gcb);
      mask TypeOptions PLCVarStartHoldPortIndex: 1 | 2 | 3 | 4 | 5 | 6 | 7 | 8 | 9 | 10 | 11 | 12 | 13 | 14 | 15 | 16 | 17 | 18 | 19 | 20 | 21 | 22 | 23 | 24 | 25 | 26 | 27 | 28 | 29 | 30 | 31 | 32 | 33 | 34 | 35 | 36 | 37 | 38 | 39 | 40 | 41 | 42 | 43 | 44 | 45 | 46 | 47 | 48 | 49 | 50 | 51 | 52 | 53 | 54 | 55 | 56 | 57 | 58 | 59
      mask TypeOptions PLCVarTScope: Local | External
      mask Callback PLCVarTScope: slplc.callbacks.updatePOUVarSS(gcb);
      mask TypeOptions PLCVarTPortType: Hidden | Inport | Outport
      mask Callback PLCVarTPortType: slplc.callbacks.updatePOUVarSS(gcb);
      mask TypeOptions PLCVarTPortIndex: 1 | 2 | 3 | 4 | 5 | 6 | 7 | 8 | 9 | 10 | 11 | 12 | 13 | 14 | 15 | 16 | 17 | 18 | 19 | 20 | 21 | 22 | 23 | 24 | 25 | 26 | 27 | 28 | 29 | 30 | 31 | 32 | 33 | 34 | 35 | 36 | 37 | 38 | 39 | 40 | 41 | 42 | 43 | 44 | 45 | 46 | 47 | 48 | 49 | 50 | 51 | 52 | 53 | 54 | 55 | 56 | 57 | 58 | 59
      mask TypeOptions PLCVarTempS1HScope: Local | External
      mask Callback PLCVarTempS1HScope: slplc.callbacks.updatePOUVarSS(gcb);
      mask TypeOptions PLCVarTempS1HPortType: Hidden | Inport | Outport
      mask Callback PLCVarTempS1HPortType: slplc.callbacks.updatePOUVarSS(gcb);
      mask TypeOptions PLCVarTempS1HPortIndex: 1 | 2 | 3 | 4 | 5 | 6 | 7 | 8 | 9 | 10 | 11 | 12 | 13 | 14 | 15 | 16 | 17 | 18 | 19 | 20 | 21 | 22 | 23 | 24 | 25 | 26 | 27 | 28 | 29 | 30 | 31 | 32 | 33 | 34 | 35 | 36 | 37 | 38 | 39 | 40 | 41 | 42 | 43 | 44 | 45 | 46 | 47 | 48 | 49 | 50 | 51 | 52 | 53 | 54 | 55 | 56 | 57 | 58 | 59
      mask TypeOptions PLCVarTempS1HDownScope: Local | External
      mask Callback PLCVarTempS1HDownScope: slplc.callbacks.updatePOUVarSS(gcb);
      mask TypeOptions PLCVarTempS1HDownPortType: Hidden | Inport | Outport
      mask Callback PLCVarTempS1HDownPortType: slplc.callbacks.updatePOUVarSS(gcb);
      mask TypeOptions PLCVarTempS1HDownPortIndex: 1 | 2 | 3 | 4 | 5 | 6 | 7 | 8 | 9 | 10 | 11 | 12 | 13 | 14 | 15 | 16 | 17 | 18 | 19 | 20 | 21 | 22 | 23 | 24 | 25 | 26 | 27 | 28 | 29 | 30 | 31 | 32 | 33 | 34 | 35 | 36 | 37 | 38 | 39 | 40 | 41 | 42 | 43 | 44 | 45 | 46 | 47 | 48 | 49 | 50 | 51 | 52 | 53 | 54 | 55 | 56 | 57 | 58 | 59
      mask TypeOptions PLCVarTempS1HUpScope: Local | External
      mask Callback PLCVarTempS1HUpScope: slplc.callbacks.updatePOUVarSS(gcb);
      mask TypeOptions PLCVarTempS1HUpPortType: Hidden | Inport | Outport
      mask Callback PLCVarTempS1HUpPortType: slplc.callbacks.updatePOUVarSS(gcb);
      mask TypeOptions PLCVarTempS1HUpPortIndex: 1 | 2 | 3 | 4 | 5 | 6 | 7 | 8 | 9 | 10 | 11 | 12 | 13 | 14 | 15 | 16 | 17 | 18 | 19 | 20 | 21 | 22 | 23 | 24 | 25 | 26 | 27 | 28 | 29 | 30 | 31 | 32 | 33 | 34 | 35 | 36 | 37 | 38 | 39 | 40 | 41 | 42 | 43 | 44 | 45 | 46 | 47 | 48 | 49 | 50 | 51 | 52 | 53 | 54 | 55 | 56 | 57 | 58 | 59
      mask TypeOptions PLCVarTempS1HupScope: Local | External
      mask Callback PLCVarTempS1HupScope: slplc.callbacks.updatePOUVarSS(gcb);
      mask TypeOptions PLCVarTempS1HupPortType: Hidden | Inport | Outport
      mask Callback PLCVarTempS1HupPortType: slplc.callbacks.updatePOUVarSS(gcb);
      mask TypeOptions PLCVarTempS1HupPortIndex: 1 | 2 | 3 | 4 | 5 | 6 | 7 | 8 | 9 | 10 | 11 | 12 | 13 | 14 | 15 | 16 | 17 | 18 | 19 | 20 | 21 | 22 | 23 | 24 | 25 | 26 | 27 | 28 | 29 | 30 | 31 | 32 | 33 | 34 | 35 | 36 | 37 | 38 | 39 | 40 | 41 | 42 | 43 | 44 | 45 | 46 | 47 | 48 | 49 | 50 | 51 | 52 | 53 | 54 | 55 | 56 | 57 | 58 | 59
      mask TypeOptions PLCVarTempS2HScope: Local | External
      mask Callback PLCVarTempS2HScope: slplc.callbacks.updatePOUVarSS(gcb);
      mask TypeOptions PLCVarTempS2HPortType: Hidden | Inport | Outport
      mask Callback PLCVarTempS2HPortType: slplc.callbacks.updatePOUVarSS(gcb);
      mask TypeOptions PLCVarTempS2HPortIndex: 1 | 2 | 3 | 4 | 5 | 6 | 7 | 8 | 9 | 10 | 11 | 12 | 13 | 14 | 15 | 16 | 17 | 18 | 19 | 20 | 21 | 22 | 23 | 24 | 25 | 26 | 27 | 28 | 29 | 30 | 31 | 32 | 33 | 34 | 35 | 36 | 37 | 38 | 39 | 40 | 41 | 42 | 43 | 44 | 45 | 46 | 47 | 48 | 49 | 50 | 51 | 52 | 53 | 54 | 55 | 56 | 57 | 58 | 59
      mask TypeOptions PLCVarTempS2HDownScope: Local | External
      mask Callback PLCVarTempS2HDownScope: slplc.callbacks.updatePOUVarSS(gcb);
      mask TypeOptions PLCVarTempS2HDownPortType: Hidden | Inport | Outport
      mask Callback PLCVarTempS2HDownPortType: slplc.callbacks.updatePOUVarSS(gcb);
      mask TypeOptions PLCVarTempS2HDownPortIndex: 1 | 2 | 3 | 4 | 5 | 6 | 7 | 8 | 9 | 10 | 11 | 12 | 13 | 14 | 15 | 16 | 17 | 18 | 19 | 20 | 21 | 22 | 23 | 24 | 25 | 26 | 27 | 28 | 29 | 30 | 31 | 32 | 33 | 34 | 35 | 36 | 37 | 38 | 39 | 40 | 41 | 42 | 43 | 44 | 45 | 46 | 47 | 48 | 49 | 50 | 51 | 52 | 53 | 54 | 55 | 56 | 57 | 58 | 59
      mask TypeOptions PLCVarTempS2HUpScope: Local | External
      mask Callback PLCVarTempS2HUpScope: slplc.callbacks.updatePOUVarSS(gcb);
      mask TypeOptions PLCVarTempS2HUpPortType: Hidden | Inport | Outport
      mask Callback PLCVarTempS2HUpPortType: slplc.callbacks.updatePOUVarSS(gcb);
      mask TypeOptions PLCVarTempS2HUpPortIndex: 1 | 2 | 3 | 4 | 5 | 6 | 7 | 8 | 9 | 10 | 11 | 12 | 13 | 14 | 15 | 16 | 17 | 18 | 19 | 20 | 21 | 22 | 23 | 24 | 25 | 26 | 27 | 28 | 29 | 30 | 31 | 32 | 33 | 34 | 35 | 36 | 37 | 38 | 39 | 40 | 41 | 42 | 43 | 44 | 45 | 46 | 47 | 48 | 49 | 50 | 51 | 52 | 53 | 54 | 55 | 56 | 57 | 58 | 59
      mask TypeOptions PLCVarTempS2LScope: Local | External
      mask Callback PLCVarTempS2LScope: slplc.callbacks.updatePOUVarSS(gcb);
      mask TypeOptions PLCVarTempS2LPortType: Hidden | Inport | Outport
      mask Callback PLCVarTempS2LPortType: slplc.callbacks.updatePOUVarSS(gcb);
      mask TypeOptions PLCVarTempS2LPortIndex: 1 | 2 | 3 | 4 | 5 | 6 | 7 | 8 | 9 | 10 | 11 | 12 | 13 | 14 | 15 | 16 | 17 | 18 | 19 | 20 | 21 | 22 | 23 | 24 | 25 | 26 | 27 | 28 | 29 | 30 | 31 | 32 | 33 | 34 | 35 | 36 | 37 | 38 | 39 | 40 | 41 | 42 | 43 | 44 | 45 | 46 | 47 | 48 | 49 | 50 | 51 | 52 | 53 | 54 | 55 | 56 | 57 | 58 | 59
      mask TypeOptions PLCVarTempS2LDownScope: Local | External
      mask Callback PLCVarTempS2LDownScope: slplc.callbacks.updatePOUVarSS(gcb);
      mask TypeOptions PLCVarTempS2LDownPortType: Hidden | Inport | Outport
      mask Callback PLCVarTempS2LDownPortType: slplc.callbacks.updatePOUVarSS(gcb);
      mask TypeOptions PLCVarTempS2LDownPortIndex: 1 | 2 | 3 | 4 | 5 | 6 | 7 | 8 | 9 | 10 | 11 | 12 | 13 | 14 | 15 | 16 | 17 | 18 | 19 | 20 | 21 | 22 | 23 | 24 | 25 | 26 | 27 | 28 | 29 | 30 | 31 | 32 | 33 | 34 | 35 | 36 | 37 | 38 | 39 | 40 | 41 | 42 | 43 | 44 | 45 | 46 | 47 | 48 | 49 | 50 | 51 | 52 | 53 | 54 | 55 | 56 | 57 | 58 | 59
      mask TypeOptions PLCVarTempS2LUpScope: Local | External
      mask Callback PLCVarTempS2LUpScope: slplc.callbacks.updatePOUVarSS(gcb);
      mask TypeOptions PLCVarTempS2LUpPortType: Hidden | Inport | Outport
      mask Callback PLCVarTempS2LUpPortType: slplc.callbacks.updatePOUVarSS(gcb);
      mask TypeOptions PLCVarTempS2LUpPortIndex: 1 | 2 | 3 | 4 | 5 | 6 | 7 | 8 | 9 | 10 | 11 | 12 | 13 | 14 | 15 | 16 | 17 | 18 | 19 | 20 | 21 | 22 | 23 | 24 | 25 | 26 | 27 | 28 | 29 | 30 | 31 | 32 | 33 | 34 | 35 | 36 | 37 | 38 | 39 | 40 | 41 | 42 | 43 | 44 | 45 | 46 | 47 | 48 | 49 | 50 | 51 | 52 | 53 | 54 | 55 | 56 | 57 | 58 | 59
      mask TypeOptions PLCVarTempS3LScope: Local | External
      mask Callback PLCVarTempS3LScope: slplc.callbacks.updatePOUVarSS(gcb);
      mask TypeOptions PLCVarTempS3LPortType: Hidden | Inport | Outport
      mask Callback PLCVarTempS3LPortType: slplc.callbacks.updatePOUVarSS(gcb);
      mask TypeOptions PLCVarTempS3LPortIndex: 1 | 2 | 3 | 4 | 5 | 6 | 7 | 8 | 9 | 10 | 11 | 12 | 13 | 14 | 15 | 16 | 17 | 18 | 19 | 20 | 21 | 22 | 23 | 24 | 25 | 26 | 27 | 28 | 29 | 30 | 31 | 32 | 33 | 34 | 35 | 36 | 37 | 38 | 39 | 40 | 41 | 42 | 43 | 44 | 45 | 46 | 47 | 48 | 49 | 50 | 51 | 52 | 53 | 54 | 55 | 56 | 57 | 58 | 59
      mask TypeOptions PLCVarTempS3LDownScope: Local | External
      mask Callback PLCVarTempS3LDownScope: slplc.callbacks.updatePOUVarSS(gcb);
      mask TypeOptions PLCVarTempS3LDownPortType: Hidden | Inport | Outport
      mask Callback PLCVarTempS3LDownPortType: slplc.callbacks.updatePOUVarSS(gcb);
      mask TypeOptions PLCVarTempS3LDownPortIndex: 1 | 2 | 3 | 4 | 5 | 6 | 7 | 8 | 9 | 10 | 11 | 12 | 13 | 14 | 15 | 16 | 17 | 18 | 19 | 20 | 21 | 22 | 23 | 24 | 25 | 26 | 27 | 28 | 29 | 30 | 31 | 32 | 33 | 34 | 35 | 36 | 37 | 38 | 39 | 40 | 41 | 42 | 43 | 44 | 45 | 46 | 47 | 48 | 49 | 50 | 51 | 52 | 53 | 54 | 55 | 56 | 57 | 58 | 59
      mask TypeOptions PLCVarTempS3LUpScope: Local | External
      mask Callback PLCVarTempS3LUpScope: slplc.callbacks.updatePOUVarSS(gcb);
      mask TypeOptions PLCVarTempS3LUpPortType: Hidden | Inport | Outport
      mask Callback PLCVarTempS3LUpPortType: slplc.callbacks.updatePOUVarSS(gcb);
      mask TypeOptions PLCVarTempS3LUpPortIndex: 1 | 2 | 3 | 4 | 5 | 6 | 7 | 8 | 9 | 10 | 11 | 12 | 13 | 14 | 15 | 16 | 17 | 18 | 19 | 20 | 21 | 22 | 23 | 24 | 25 | 26 | 27 | 28 | 29 | 30 | 31 | 32 | 33 | 34 | 35 | 36 | 37 | 38 | 39 | 40 | 41 | 42 | 43 | 44 | 45 | 46 | 47 | 48 | 49 | 50 | 51 | 52 | 53 | 54 | 55 | 56 | 57 | 58 | 59
      mask TypeOptions PLCVarVARVELScope: Local | External
      mask Callback PLCVarVARVELScope: slplc.callbacks.updatePOUVarSS(gcb);
      mask TypeOptions PLCVarVARVELPortType: Hidden | Inport | Outport
      mask Callback PLCVarVARVELPortType: slplc.callbacks.updatePOUVarSS(gcb);
      mask TypeOptions PLCVarVARVELPortIndex: 1 | 2 | 3 | 4 | 5 | 6 | 7 | 8 | 9 | 10 | 11 | 12 | 13 | 14 | 15 | 16 | 17 | 18 | 19 | 20 | 21 | 22 | 23 | 24 | 25 | 26 | 27 | 28 | 29 | 30 | 31 | 32 | 33 | 34 | 35 | 36 | 37 | 38 | 39 | 40 | 41 | 42 | 43 | 44 | 45 | 46 | 47 | 48 | 49 | 50 | 51 | 52 | 53 | 54 | 55 | 56 | 57 | 58 | 59
      mask TypeOptions PLCVarF1PBScope: Local | External
      mask Callback PLCVarF1PBScope: slplc.callbacks.updatePOUVarSS(gcb);
      mask TypeOptions PLCVarF1PBPortType: Hidden | Inport | Outport
      mask Callback PLCVarF1PBPortType: slplc.callbacks.updatePOUVarSS(gcb);
      mask TypeOptions PLCVarF1PBPortIndex: 1 | 2 | 3 | 4 | 5 | 6 | 7 | 8 | 9 | 10 | 11 | 12 | 13 | 14 | 15 | 16 | 17 | 18 | 19 | 20 | 21 | 22 | 23 | 24 | 25 | 26 | 27 | 28 | 29 | 30 | 31 | 32 | 33 | 34 | 35 | 36 | 37 | 38 | 39 | 40 | 41 | 42 | 43 | 44 | 45 | 46 | 47 | 48 | 49 | 50 | 51 | 52 | 53 | 54 | 55 | 56 | 57 | 58 | 59
      mask TypeOptions PLCVarF1UpBScope: Local | External
      mask Callback PLCVarF1UpBScope: slplc.callbacks.updatePOUVarSS(gcb);
      mask TypeOptions PLCVarF1UpBPortType: Hidden | Inport | Outport
      mask Callback PLCVarF1UpBPortType: slplc.callbacks.updatePOUVarSS(gcb);
      mask TypeOptions PLCVarF1UpBPortIndex: 1 | 2 | 3 | 4 | 5 | 6 | 7 | 8 | 9 | 10 | 11 | 12 | 13 | 14 | 15 | 16 | 17 | 18 | 19 | 20 | 21 | 22 | 23 | 24 | 25 | 26 | 27 | 28 | 29 | 30 | 31 | 32 | 33 | 34 | 35 | 36 | 37 | 38 | 39 | 40 | 41 | 42 | 43 | 44 | 45 | 46 | 47 | 48 | 49 | 50 | 51 | 52 | 53 | 54 | 55 | 56 | 57 | 58 | 59
      mask TypeOptions PLCVarF2DownBScope: Local | External
      mask Callback PLCVarF2DownBScope: slplc.callbacks.updatePOUVarSS(gcb);
      mask TypeOptions PLCVarF2DownBPortType: Hidden | Inport | Outport
      mask Callback PLCVarF2DownBPortType: slplc.callbacks.updatePOUVarSS(gcb);
      mask TypeOptions PLCVarF2DownBPortIndex: 1 | 2 | 3 | 4 | 5 | 6 | 7 | 8 | 9 | 10 | 11 | 12 | 13 | 14 | 15 | 16 | 17 | 18 | 19 | 20 | 21 | 22 | 23 | 24 | 25 | 26 | 27 | 28 | 29 | 30 | 31 | 32 | 33 | 34 | 35 | 36 | 37 | 38 | 39 | 40 | 41 | 42 | 43 | 44 | 45 | 46 | 47 | 48 | 49 | 50 | 51 | 52 | 53 | 54 | 55 | 56 | 57 | 58 | 59
      mask TypeOptions PLCVarF2PBScope: Local | External
      mask Callback PLCVarF2PBScope: slplc.callbacks.updatePOUVarSS(gcb);
      mask TypeOptions PLCVarF2PBPortType: Hidden | Inport | Outport
      mask Callback PLCVarF2PBPortType: slplc.callbacks.updatePOUVarSS(gcb);
      mask TypeOptions PLCVarF2PBPortIndex: 1 | 2 | 3 | 4 | 5 | 6 | 7 | 8 | 9 | 10 | 11 | 12 | 13 | 14 | 15 | 16 | 17 | 18 | 19 | 20 | 21 | 22 | 23 | 24 | 25 | 26 | 27 | 28 | 29 | 30 | 31 | 32 | 33 | 34 | 35 | 36 | 37 | 38 | 39 | 40 | 41 | 42 | 43 | 44 | 45 | 46 | 47 | 48 | 49 | 50 | 51 | 52 | 53 | 54 | 55 | 56 | 57 | 58 | 59
      mask TypeOptions PLCVarF2UpBScope: Local | External
      mask Callback PLCVarF2UpBScope: slplc.callbacks.updatePOUVarSS(gcb);
      mask TypeOptions PLCVarF2UpBPortType: Hidden | Inport | Outport
      mask Callback PLCVarF2UpBPortType: slplc.callbacks.updatePOUVarSS(gcb);
      mask TypeOptions PLCVarF2UpBPortIndex: 1 | 2 | 3 | 4 | 5 | 6 | 7 | 8 | 9 | 10 | 11 | 12 | 13 | 14 | 15 | 16 | 17 | 18 | 19 | 20 | 21 | 22 | 23 | 24 | 25 | 26 | 27 | 28 | 29 | 30 | 31 | 32 | 33 | 34 | 35 | 36 | 37 | 38 | 39 | 40 | 41 | 42 | 43 | 44 | 45 | 46 | 47 | 48 | 49 | 50 | 51 | 52 | 53 | 54 | 55 | 56 | 57 | 58 | 59
      mask TypeOptions PLCVarF3DownBScope: Local | External
      mask Callback PLCVarF3DownBScope: slplc.callbacks.updatePOUVarSS(gcb);
      mask TypeOptions PLCVarF3DownBPortType: Hidden | Inport | Outport
      mask Callback PLCVarF3DownBPortType: slplc.callbacks.updatePOUVarSS(gcb);
      mask TypeOptions PLCVarF3DownBPortIndex: 1 | 2 | 3 | 4 | 5 | 6 | 7 | 8 | 9 | 10 | 11 | 12 | 13 | 14 | 15 | 16 | 17 | 18 | 19 | 20 | 21 | 22 | 23 | 24 | 25 | 26 | 27 | 28 | 29 | 30 | 31 | 32 | 33 | 34 | 35 | 36 | 37 | 38 | 39 | 40 | 41 | 42 | 43 | 44 | 45 | 46 | 47 | 48 | 49 | 50 | 51 | 52 | 53 | 54 | 55 | 56 | 57 | 58 | 59
      mask TypeOptions PLCVarF3PBScope: Local | External
      mask Callback PLCVarF3PBScope: slplc.callbacks.updatePOUVarSS(gcb);
      mask TypeOptions PLCVarF3PBPortType: Hidden | Inport | Outport
      mask Callback PLCVarF3PBPortType: slplc.callbacks.updatePOUVarSS(gcb);
      mask TypeOptions PLCVarF3PBPortIndex: 1 | 2 | 3 | 4 | 5 | 6 | 7 | 8 | 9 | 10 | 11 | 12 | 13 | 14 | 15 | 16 | 17 | 18 | 19 | 20 | 21 | 22 | 23 | 24 | 25 | 26 | 27 | 28 | 29 | 30 | 31 | 32 | 33 | 34 | 35 | 36 | 37 | 38 | 39 | 40 | 41 | 42 | 43 | 44 | 45 | 46 | 47 | 48 | 49 | 50 | 51 | 52 | 53 | 54 | 55 | 56 | 57 | 58 | 59
      mask TypeOptions PLCVarFLOOROUTScope: Local | External
      mask Callback PLCVarFLOOROUTScope: slplc.callbacks.updatePOUVarSS(gcb);
      mask TypeOptions PLCVarFLOOROUTPortType: Hidden | Inport | Outport
      mask Callback PLCVarFLOOROUTPortType: slplc.callbacks.updatePOUVarSS(gcb);
      mask TypeOptions PLCVarFLOOROUTPortIndex: 1 | 2 | 3 | 4 | 5 | 6 | 7 | 8 | 9 | 10 | 11 | 12 | 13 | 14 | 15 | 16 | 17 | 18 | 19 | 20 | 21 | 22 | 23 | 24 | 25 | 26 | 27 | 28 | 29 | 30 | 31 | 32 | 33 | 34 | 35 | 36 | 37 | 38 | 39 | 40 | 41 | 42 | 43 | 44 | 45 | 46 | 47 | 48 | 49 | 50 | 51 | 52 | 53 | 54 | 55 | 56 | 57 | 58 | 59
      mask TypeOptions PLCVarS1HScope: Local | External
      mask Callback PLCVarS1HScope: slplc.callbacks.updatePOUVarSS(gcb);
      mask TypeOptions PLCVarS1HPortType: Hidden | Inport | Outport
      mask Callback PLCVarS1HPortType: slplc.callbacks.updatePOUVarSS(gcb);
      mask TypeOptions PLCVarS1HPortIndex: 1 | 2 | 3 | 4 | 5 | 6 | 7 | 8 | 9 | 10 | 11 | 12 | 13 | 14 | 15 | 16 | 17 | 18 | 19 | 20 | 21 | 22 | 23 | 24 | 25 | 26 | 27 | 28 | 29 | 30 | 31 | 32 | 33 | 34 | 35 | 36 | 37 | 38 | 39 | 40 | 41 | 42 | 43 | 44 | 45 | 46 | 47 | 48 | 49 | 50 | 51 | 52 | 53 | 54 | 55 | 56 | 57 | 58 | 59
      mask TypeOptions PLCVarS2HScope: Local | External
      mask Callback PLCVarS2HScope: slplc.callbacks.updatePOUVarSS(gcb);
      mask TypeOptions PLCVarS2HPortType: Hidden | Inport | Outport
      mask Callback PLCVarS2HPortType: slplc.callbacks.updatePOUVarSS(gcb);
      mask TypeOptions PLCVarS2HPortIndex: 1 | 2 | 3 | 4 | 5 | 6 | 7 | 8 | 9 | 10 | 11 | 12 | 13 | 14 | 15 | 16 | 17 | 18 | 19 | 20 | 21 | 22 | 23 | 24 | 25 | 26 | 27 | 28 | 29 | 30 | 31 | 32 | 33 | 34 | 35 | 36 | 37 | 38 | 39 | 40 | 41 | 42 | 43 | 44 | 45 | 46 | 47 | 48 | 49 | 50 | 51 | 52 | 53 | 54 | 55 | 56 | 57 | 58 | 59
      mask TypeOptions PLCVarS2LScope: Local | External
      mask Callback PLCVarS2LScope: slplc.callbacks.updatePOUVarSS(gcb);
      mask TypeOptions PLCVarS2LPortType: Hidden | Inport | Outport
      mask Callback PLCVarS2LPortType: slplc.callbacks.updatePOUVarSS(gcb);
      mask TypeOptions PLCVarS2LPortIndex: 1 | 2 | 3 | 4 | 5 | 6 | 7 | 8 | 9 | 10 | 11 | 12 | 13 | 14 | 15 | 16 | 17 | 18 | 19 | 20 | 21 | 22 | 23 | 24 | 25 | 26 | 27 | 28 | 29 | 30 | 31 | 32 | 33 | 34 | 35 | 36 | 37 | 38 | 39 | 40 | 41 | 42 | 43 | 44 | 45 | 46 | 47 | 48 | 49 | 50 | 51 | 52 | 53 | 54 | 55 | 56 | 57 | 58 | 59
      mask TypeOptions PLCVarS3LScope: Local | External
      mask Callback PLCVarS3LScope: slplc.callbacks.updatePOUVarSS(gcb);
      mask TypeOptions PLCVarS3LPortType: Hidden | Inport | Outport
      mask Callback PLCVarS3LPortType: slplc.callbacks.updatePOUVarSS(gcb);
      mask TypeOptions PLCVarS3LPortIndex: 1 | 2 | 3 | 4 | 5 | 6 | 7 | 8 | 9 | 10 | 11 | 12 | 13 | 14 | 15 | 16 | 17 | 18 | 19 | 20 | 21 | 22 | 23 | 24 | 25 | 26 | 27 | 28 | 29 | 30 | 31 | 32 | 33 | 34 | 35 | 36 | 37 | 38 | 39 | 40 | 41 | 42 | 43 | 44 | 45 | 46 | 47 | 48 | 49 | 50 | 51 | 52 | 53 | 54 | 55 | 56 | 57 | 58 | 59
      mask TypeOptions PLCVarStartScope: Local | External
      mask Callback PLCVarStartScope: slplc.callbacks.updatePOUVarSS(gcb);
      mask TypeOptions PLCVarStartPortType: Hidden | Inport | Outport
      mask Callback PLCVarStartPortType: slplc.callbacks.updatePOUVarSS(gcb);
      mask TypeOptions PLCVarStartPortIndex: 1 | 2 | 3 | 4 | 5 | 6 | 7 | 8 | 9 | 10 | 11 | 12 | 13 | 14 | 15 | 16 | 17 | 18 | 19 | 20 | 21 | 22 | 23 | 24 | 25 | 26 | 27 | 28 | 29 | 30 | 31 | 32 | 33 | 34 | 35 | 36 | 37 | 38 | 39 | 40 | 41 | 42 | 43 | 44 | 45 | 46 | 47 | 48 | 49 | 50 | 51 | 52 | 53 | 54 | 55 | 56 | 57 | 58 | 59
      mask TypeOptions PLCVarStopScope: Local | External
      mask Callback PLCVarStopScope: slplc.callbacks.updatePOUVarSS(gcb);
      mask TypeOptions PLCVarStopPortType: Hidden | Inport | Outport
      mask Callback PLCVarStopPortType: slplc.callbacks.updatePOUVarSS(gcb);
      mask TypeOptions PLCVarStopPortIndex: 1 | 2 | 3 | 4 | 5 | 6 | 7 | 8 | 9 | 10 | 11 | 12 | 13 | 14 | 15 | 16 | 17 | 18 | 19 | 20 | 21 | 22 | 23 | 24 | 25 | 26 | 27 | 28 | 29 | 30 | 31 | 32 | 33 | 34 | 35 | 36 | 37 | 38 | 39 | 40 | 41 | 42 | 43 | 44 | 45 | 46 | 47 | 48 | 49 | 50 | 51 | 52 | 53 | 54 | 55 | 56 | 57 | 58 | 59
      mask TypeOptions PLCVarVELOUTScope: Local | External
      mask Callback PLCVarVELOUTScope: slplc.callbacks.updatePOUVarSS(gcb);
      mask TypeOptions PLCVarVELOUTPortType: Hidden | Inport | Outport
      mask Callback PLCVarVELOUTPortType: slplc.callbacks.updatePOUVarSS(gcb);
      mask TypeOptions PLCVarVELOUTPortIndex: 1 | 2 | 3 | 4 | 5 | 6 | 7 | 8 | 9 | 10 | 11 | 12 | 13 | 14 | 15 | 16 | 17 | 18 | 19 | 20 | 21 | 22 | 23 | 24 | 25 | 26 | 27 | 28 | 29 | 30 | 31 | 32 | 33 | 34 | 35 | 36 | 37 | 38 | 39 | 40 | 41 | 42 | 43 | 44 | 45 | 46 | 47 | 48 | 49 | 50 | 51 | 52 | 53 | 54 | 55 | 56 | 57 | 58 | 59
      mask DialogControl PLCBlockTitle Prompt: Program Variable Spreadsheet
      mask DialogControl PLCVarListHeaderName Prompt: Name
      mask DialogControl PLCVarListHeaderScope Prompt: Scope
      mask DialogControl PLCVarListHeaderDataType Prompt: Data Type
      mask DialogControl PLCVarListHeaderSize Prompt: Size
      mask DialogControl PLCVarListHeaderInitialValue Prompt: Initial Value
      mask DialogControl PLCVarListHeaderToDelete Prompt: Delete
  Rung Terminal : Subsystem  Priority=118  DisableCoverage=on  TreatAsAtomicUnit=on  mask{PLCRungTerminalIndex=16, PLCBlockType=RungTerminal}
      settings: AttributesFormatString=Rung %<PLCRungTerminalIndex>
      mask Help: web([docroot '/plccoder/ref/rungterminal' '.html']);
      mask DialogControl PLCBlockTitle Prompt: Rung Terminal
      mask DialogControl PLCBlockDescText Prompt: This is the ladder diagram rung terminal.
  Rung Terminal1 : Subsystem  Priority=7  DisableCoverage=on  TreatAsAtomicUnit=on  mask{PLCRungTerminalIndex=1, PLCBlockType=RungTerminal}
      settings: AttributesFormatString=Rung %<PLCRungTerminalIndex>
      mask Help: web([docroot '/plccoder/ref/rungterminal' '.html']);
      mask DialogControl PLCBlockTitle Prompt: Rung Terminal
      mask DialogControl PLCBlockDescText Prompt: This is the ladder diagram rung terminal.
  Rung Terminal10 : Subsystem  Priority=168  DisableCoverage=on  TreatAsAtomicUnit=on  mask{PLCRungTerminalIndex=22, PLCBlockType=RungTerminal}
      settings: AttributesFormatString=Rung %<PLCRungTerminalIndex>
      mask Help: web([docroot '/plccoder/ref/rungterminal' '.html']);
      mask DialogControl PLCBlockTitle Prompt: Rung Terminal
      mask DialogControl PLCBlockDescText Prompt: This is the ladder diagram rung terminal.
  Rung Terminal11 : Subsystem  Priority=181  DisableCoverage=on  TreatAsAtomicUnit=on  mask{PLCRungTerminalIndex=23, PLCBlockType=RungTerminal}
      settings: AttributesFormatString=Rung %<PLCRungTerminalIndex>
      mask Help: web([docroot '/plccoder/ref/rungterminal' '.html']);
      mask DialogControl PLCBlockTitle Prompt: Rung Terminal
      mask DialogControl PLCBlockDescText Prompt: This is the ladder diagram rung terminal.
  Rung Terminal12 : Subsystem  Priority=254  DisableCoverage=on  TreatAsAtomicUnit=on  mask{PLCRungTerminalIndex=32, PLCBlockType=RungTerminal}
      settings: AttributesFormatString=Rung %<PLCRungTerminalIndex>
      mask Help: web([docroot '/plccoder/ref/rungterminal' '.html']);
      mask DialogControl PLCBlockTitle Prompt: Rung Terminal
      mask DialogControl PLCBlockDescText Prompt: This is the ladder diagram rung terminal.
  Rung Terminal13 : Subsystem  Priority=244  DisableCoverage=on  TreatAsAtomicUnit=on  mask{PLCRungTerminalIndex=30, PLCBlockType=RungTerminal}
      settings: AttributesFormatString=Rung %<PLCRungTerminalIndex>
      mask Help: web([docroot '/plccoder/ref/rungterminal' '.html']);
      mask DialogControl PLCBlockTitle Prompt: Rung Terminal
      mask DialogControl PLCBlockDescText Prompt: This is the ladder diagram rung terminal.
  Rung Terminal14 : Subsystem  Priority=262  DisableCoverage=on  TreatAsAtomicUnit=on  mask{PLCRungTerminalIndex=33, PLCBlockType=RungTerminal}
      settings: AttributesFormatString=Rung %<PLCRungTerminalIndex>
      mask Help: web([docroot '/plccoder/ref/rungterminal' '.html']);
      mask DialogControl PLCBlockTitle Prompt: Rung Terminal
      mask DialogControl PLCBlockDescText Prompt: This is the ladder diagram rung terminal.
  Rung Terminal15 : Subsystem  Priority=87  DisableCoverage=on  TreatAsAtomicUnit=on  mask{PLCRungTerminalIndex=12, PLCBlockType=RungTerminal}
      settings: AttributesFormatString=Rung %<PLCRungTerminalIndex>
      mask Help: web([docroot '/plccoder/ref/rungterminal' '.html']);
      mask DialogControl PLCBlockTitle Prompt: Rung Terminal
      mask DialogControl PLCBlockDescText Prompt: This is the ladder diagram rung terminal.
  Rung Terminal16 : Subsystem  Priority=80  DisableCoverage=on  TreatAsAtomicUnit=on  mask{PLCRungTerminalIndex=11, PLCBlockType=RungTerminal}
      settings: AttributesFormatString=Rung %<PLCRungTerminalIndex>
      mask Help: web([docroot '/plccoder/ref/rungterminal' '.html']);
      mask DialogControl PLCBlockTitle Prompt: Rung Terminal
      mask DialogControl PLCBlockDescText Prompt: This is the ladder diagram rung terminal.
  Rung Terminal17 : Subsystem  Priority=70  DisableCoverage=on  TreatAsAtomicUnit=on  mask{PLCRungTerminalIndex=10, PLCBlockType=RungTerminal}
      settings: AttributesFormatString=Rung %<PLCRungTerminalIndex>
      mask Help: web([docroot '/plccoder/ref/rungterminal' '.html']);
      mask DialogControl PLCBlockTitle Prompt: Rung Terminal
      mask DialogControl PLCBlockDescText Prompt: This is the ladder diagram rung terminal.
  Rung Terminal18 : Subsystem  Priority=111  DisableCoverage=on  TreatAsAtomicUnit=on  mask{PLCRungTerminalIndex=15, PLCBlockType=RungTerminal}
      settings: AttributesFormatString=Rung %<PLCRungTerminalIndex>
      mask Help: web([docroot '/plccoder/ref/rungterminal' '.html']);
      mask DialogControl PLCBlockTitle Prompt: Rung Terminal
      mask DialogControl PLCBlockDescText Prompt: This is the ladder diagram rung terminal.
  Rung Terminal19 : Subsystem  Priority=103  DisableCoverage=on  TreatAsAtomicUnit=on  mask{PLCRungTerminalIndex=14, PLCBlockType=RungTerminal}
      settings: AttributesFormatString=Rung %<PLCRungTerminalIndex>
      mask Help: web([docroot '/plccoder/ref/rungterminal' '.html']);
      mask DialogControl PLCBlockTitle Prompt: Rung Terminal
      mask DialogControl PLCBlockDescText Prompt: This is the ladder diagram rung terminal.
  Rung Terminal2 : Subsystem  Priority=125  DisableCoverage=on  TreatAsAtomicUnit=on  mask{PLCRungTerminalIndex=17, PLCBlockType=RungTerminal}
      settings: AttributesFormatString=Rung %<PLCRungTerminalIndex>
      mask Help: web([docroot '/plccoder/ref/rungterminal' '.html']);
      mask DialogControl PLCBlockTitle Prompt: Rung Terminal
      mask DialogControl PLCBlockDescText Prompt: This is the ladder diagram rung terminal.
  Rung Terminal20 : Subsystem  Priority=95  DisableCoverage=on  TreatAsAtomicUnit=on  mask{PLCRungTerminalIndex=13, PLCBlockType=RungTerminal}
      settings: AttributesFormatString=Rung %<PLCRungTerminalIndex>
      mask Help: web([docroot '/plccoder/ref/rungterminal' '.html']);
      mask DialogControl PLCBlockTitle Prompt: Rung Terminal
      mask DialogControl PLCBlockDescText Prompt: This is the ladder diagram rung terminal.
  Rung Terminal21 : Subsystem  Priority=42  DisableCoverage=on  TreatAsAtomicUnit=on  mask{PLCRungTerminalIndex=6, PLCBlockType=RungTerminal}
      settings: AttributesFormatString=Rung %<PLCRungTerminalIndex>
      mask Help: web([docroot '/plccoder/ref/rungterminal' '.html']);
      mask DialogControl PLCBlockTitle Prompt: Rung Terminal
      mask DialogControl PLCBlockDescText Prompt: This is the ladder diagram rung terminal.
  Rung Terminal22 : Subsystem  Priority=56  DisableCoverage=on  TreatAsAtomicUnit=on  mask{PLCRungTerminalIndex=8, PLCBlockType=RungTerminal}
      settings: AttributesFormatString=Rung %<PLCRungTerminalIndex>
      mask Help: web([docroot '/plccoder/ref/rungterminal' '.html']);
      mask DialogControl PLCBlockTitle Prompt: Rung Terminal
      mask DialogControl PLCBlockDescText Prompt: This is the ladder diagram rung terminal.
  Rung Terminal23 : Subsystem  Priority=21  DisableCoverage=on  TreatAsAtomicUnit=on  mask{PLCRungTerminalIndex=3, PLCBlockType=RungTerminal}
      settings: AttributesFormatString=Rung %<PLCRungTerminalIndex>
      mask Help: web([docroot '/plccoder/ref/rungterminal' '.html']);
      mask DialogControl PLCBlockTitle Prompt: Rung Terminal
      mask DialogControl PLCBlockDescText Prompt: This is the ladder diagram rung terminal.
  Rung Terminal24 : Subsystem  Priority=28  DisableCoverage=on  TreatAsAtomicUnit=on  mask{PLCRungTerminalIndex=4, PLCBlockType=RungTerminal}
      settings: AttributesFormatString=Rung %<PLCRungTerminalIndex>
      mask Help: web([docroot '/plccoder/ref/rungterminal' '.html']);
      mask DialogControl PLCBlockTitle Prompt: Rung Terminal
      mask DialogControl PLCBlockDescText Prompt: This is the ladder diagram rung terminal.
  Rung Terminal25 : Subsystem  Priority=63  DisableCoverage=on  TreatAsAtomicUnit=on  mask{PLCRungTerminalIndex=9, PLCBlockType=RungTerminal}
      settings: AttributesFormatString=Rung %<PLCRungTerminalIndex>
      mask Help: web([docroot '/plccoder/ref/rungterminal' '.html']);
      mask DialogControl PLCBlockTitle Prompt: Rung Terminal
      mask DialogControl PLCBlockDescText Prompt: This is the ladder diagram rung terminal.
  Rung Terminal26 : Subsystem  Priority=49  DisableCoverage=on  TreatAsAtomicUnit=on  mask{PLCRungTerminalIndex=7, PLCBlockType=RungTerminal}
      settings: AttributesFormatString=Rung %<PLCRungTerminalIndex>
      mask Help: web([docroot '/plccoder/ref/rungterminal' '.html']);
      mask DialogControl PLCBlockTitle Prompt: Rung Terminal
      mask DialogControl PLCBlockDescText Prompt: This is the ladder diagram rung terminal.
  Rung Terminal27 : Subsystem  Priority=35  DisableCoverage=on  TreatAsAtomicUnit=on  mask{PLCRungTerminalIndex=5, PLCBlockType=RungTerminal}
      settings: AttributesFormatString=Rung %<PLCRungTerminalIndex>
      mask Help: web([docroot '/plccoder/ref/rungterminal' '.html']);
      mask DialogControl PLCBlockTitle Prompt: Rung Terminal
      mask DialogControl PLCBlockDescText Prompt: This is the ladder diagram rung terminal.
  Rung Terminal28 : Subsystem  Priority=14  DisableCoverage=on  TreatAsAtomicUnit=on  mask{PLCRungTerminalIndex=2, PLCBlockType=RungTerminal}
      settings: AttributesFormatString=Rung %<PLCRungTerminalIndex>
      mask Help: web([docroot '/plccoder/ref/rungterminal' '.html']);
      mask DialogControl PLCBlockTitle Prompt: Rung Terminal
      mask DialogControl PLCBlockDescText Prompt: This is the ladder diagram rung terminal.
  Rung Terminal29 : Subsystem  Priority=188  DisableCoverage=on  TreatAsAtomicUnit=on  mask{PLCRungTerminalIndex=24, PLCBlockType=RungTerminal}
      settings: AttributesFormatString=Rung %<PLCRungTerminalIndex>
      mask Help: web([docroot '/plccoder/ref/rungterminal' '.html']);
      mask DialogControl PLCBlockTitle Prompt: Rung Terminal
      mask DialogControl PLCBlockDescText Prompt: This is the ladder diagram rung terminal.
  Rung Terminal3 : Subsystem  Priority=132  DisableCoverage=on  TreatAsAtomicUnit=on  mask{PLCRungTerminalIndex=18, PLCBlockType=RungTerminal}
      settings: AttributesFormatString=Rung %<PLCRungTerminalIndex>
      mask Help: web([docroot '/plccoder/ref/rungterminal' '.html']);
      mask DialogControl PLCBlockTitle Prompt: Rung Terminal
      mask DialogControl PLCBlockDescText Prompt: This is the ladder diagram rung terminal.
  Rung Terminal30 : Subsystem  Priority=195  DisableCoverage=on  TreatAsAtomicUnit=on  mask{PLCRungTerminalIndex=25, PLCBlockType=RungTerminal}
      settings: AttributesFormatString=Rung %<PLCRungTerminalIndex>
      mask Help: web([docroot '/plccoder/ref/rungterminal' '.html']);
      mask DialogControl PLCBlockTitle Prompt: Rung Terminal
      mask DialogControl PLCBlockDescText Prompt: This is the ladder diagram rung terminal.
  Rung Terminal31 : Subsystem  Priority=208  DisableCoverage=on  TreatAsAtomicUnit=on  mask{PLCRungTerminalIndex=27, PLCBlockType=RungTerminal}
      settings: AttributesFormatString=Rung %<PLCRungTerminalIndex>
      mask Help: web([docroot '/plccoder/ref/rungterminal' '.html']);
      mask DialogControl PLCBlockTitle Prompt: Rung Terminal
      mask DialogControl PLCBlockDescText Prompt: This is the ladder diagram rung terminal.
  Rung Terminal32 : Subsystem  Priority=290  DisableCoverage=on  TreatAsAtomicUnit=on  mask{PLCRungTerminalIndex=37, PLCBlockType=RungTerminal}
      settings: AttributesFormatString=Rung %<PLCRungTerminalIndex>
      mask Help: web([docroot '/plccoder/ref/rungterminal' '.html']);
      mask DialogControl PLCBlockTitle Prompt: Rung Terminal
      mask DialogControl PLCBlockDescText Prompt: This is the ladder diagram rung terminal.
  Rung Terminal33 : Subsystem  Priority=246  DisableCoverage=on  TreatAsAtomicUnit=on  mask{PLCRungTerminalIndex=31, PLCBlockType=RungTerminal}
      settings: AttributesFormatString=Rung %<PLCRungTerminalIndex>
      mask Help: web([docroot '/plccoder/ref/rungterminal' '.html']);
      mask DialogControl PLCBlockTitle Prompt: Rung Terminal
      mask DialogControl PLCBlockDescText Prompt: This is the ladder diagram rung terminal.
  Rung Terminal34 : Subsystem  Priority=276  DisableCoverage=on  TreatAsAtomicUnit=on  mask{PLCRungTerminalIndex=35, PLCBlockType=RungTerminal}
      settings: AttributesFormatString=Rung %<PLCRungTerminalIndex>
      mask Help: web([docroot '/plccoder/ref/rungterminal' '.html']);
      mask DialogControl PLCBlockTitle Prompt: Rung Terminal
      mask DialogControl PLCBlockDescText Prompt: This is the ladder diagram rung terminal.
  Rung Terminal35 : Subsystem  Priority=298  DisableCoverage=on  TreatAsAtomicUnit=on  mask{PLCRungTerminalIndex=38, PLCBlockType=RungTerminal}
      settings: AttributesFormatString=Rung %<PLCRungTerminalIndex>
      mask Help: web([docroot '/plccoder/ref/rungterminal' '.html']);
      mask DialogControl PLCBlockTitle Prompt: Rung Terminal
      mask DialogControl PLCBlockDescText Prompt: This is the ladder diagram rung terminal.
  Rung Terminal36 : Subsystem  Priority=269  DisableCoverage=on  TreatAsAtomicUnit=on  mask{PLCRungTerminalIndex=34, PLCBlockType=RungTerminal}
      settings: AttributesFormatString=Rung %<PLCRungTerminalIndex>
      mask Help: web([docroot '/plccoder/ref/rungterminal' '.html']);
      mask DialogControl PLCBlockTitle Prompt: Rung Terminal
      mask DialogControl PLCBlockDescText Prompt: This is the ladder diagram rung terminal.
  Rung Terminal37 : Subsystem  Priority=283  DisableCoverage=on  TreatAsAtomicUnit=on  mask{PLCRungTerminalIndex=36, PLCBlockType=RungTerminal}
      settings: AttributesFormatString=Rung %<PLCRungTerminalIndex>
      mask Help: web([docroot '/plccoder/ref/rungterminal' '.html']);
      mask DialogControl PLCBlockTitle Prompt: Rung Terminal
      mask DialogControl PLCBlockDescText Prompt: This is the ladder diagram rung terminal.
  Rung Terminal38 : Subsystem  Priority=303  DisableCoverage=on  TreatAsAtomicUnit=on  mask{PLCRungTerminalIndex=39, PLCBlockType=RungTerminal}
      settings: AttributesFormatString=Rung %<PLCRungTerminalIndex>
      mask Help: web([docroot '/plccoder/ref/rungterminal' '.html']);
      mask DialogControl PLCBlockTitle Prompt: Rung Terminal
      mask DialogControl PLCBlockDescText Prompt: This is the ladder diagram rung terminal.
  Rung Terminal39 : Subsystem  Priority=308  DisableCoverage=on  TreatAsAtomicUnit=on  mask{PLCRungTerminalIndex=40, PLCBlockType=RungTerminal}
      settings: AttributesFormatString=Rung %<PLCRungTerminalIndex>
      mask Help: web([docroot '/plccoder/ref/rungterminal' '.html']);
      mask DialogControl PLCBlockTitle Prompt: Rung Terminal
      mask DialogControl PLCBlockDescText Prompt: This is the ladder diagram rung terminal.
  Rung Terminal4 : Subsystem  Priority=139  DisableCoverage=on  TreatAsAtomicUnit=on  mask{PLCRungTerminalIndex=19, PLCBlockType=RungTerminal}
      settings: AttributesFormatString=Rung %<PLCRungTerminalIndex>
      mask Help: web([docroot '/plccoder/ref/rungterminal' '.html']);
      mask DialogControl PLCBlockTitle Prompt: Rung Terminal
      mask DialogControl PLCBlockDescText Prompt: This is the ladder diagram rung terminal.
  Rung Terminal5 : Subsystem  Priority=148  DisableCoverage=on  TreatAsAtomicUnit=on  mask{PLCRungTerminalIndex=20, PLCBlockType=RungTerminal}
      settings: AttributesFormatString=Rung %<PLCRungTerminalIndex>
      mask Help: web([docroot '/plccoder/ref/rungterminal' '.html']);
      mask DialogControl PLCBlockTitle Prompt: Rung Terminal
      mask DialogControl PLCBlockDescText Prompt: This is the ladder diagram rung terminal.
  Rung Terminal6 : Subsystem  Priority=155  DisableCoverage=on  TreatAsAtomicUnit=on  mask{PLCRungTerminalIndex=21, PLCBlockType=RungTerminal}
      settings: AttributesFormatString=Rung %<PLCRungTerminalIndex>
      mask Help: web([docroot '/plccoder/ref/rungterminal' '.html']);
      mask DialogControl PLCBlockTitle Prompt: Rung Terminal
      mask DialogControl PLCBlockDescText Prompt: This is the ladder diagram rung terminal.
  Rung Terminal7 : Subsystem  Priority=202  DisableCoverage=on  TreatAsAtomicUnit=on  mask{PLCRungTerminalIndex=26, PLCBlockType=RungTerminal}
      settings: AttributesFormatString=Rung %<PLCRungTerminalIndex>
      mask Help: web([docroot '/plccoder/ref/rungterminal' '.html']);
      mask DialogControl PLCBlockTitle Prompt: Rung Terminal
      mask DialogControl PLCBlockDescText Prompt: This is the ladder diagram rung terminal.
  Rung Terminal8 : Subsystem  Priority=232  DisableCoverage=on  TreatAsAtomicUnit=on  mask{PLCRungTerminalIndex=28, PLCBlockType=RungTerminal}
      settings: AttributesFormatString=Rung %<PLCRungTerminalIndex>
      mask Help: web([docroot '/plccoder/ref/rungterminal' '.html']);
      mask DialogControl PLCBlockTitle Prompt: Rung Terminal
      mask DialogControl PLCBlockDescText Prompt: This is the ladder diagram rung terminal.
  Rung Terminal9 : Subsystem  Priority=240  DisableCoverage=on  TreatAsAtomicUnit=on  mask{PLCRungTerminalIndex=29, PLCBlockType=RungTerminal}
      settings: AttributesFormatString=Rung %<PLCRungTerminalIndex>
      mask Help: web([docroot '/plccoder/ref/rungterminal' '.html']);
      mask DialogControl PLCBlockTitle Prompt: Rung Terminal
      mask DialogControl PLCBlockDescText Prompt: This is the ladder diagram rung terminal.
  SUB : Subsystem  Priority=288  TreatAsAtomicUnit=on  mask{PLCBlockType=SUB, PLCPOUType=stdFC}
      mask Help: web([docroot '/plccoder/ref/sub' '.html']);
      mask DialogControl PLCBlockTitle Prompt: Substract (SUB)
      mask DialogControl PLCBlockDesc Prompt: Substract Source B from Source A.
      mask Display: disp('SUB');
  TON : Subsystem  Priority=238  TreatAsAtomicUnit=on  mask{PLCOperandTag=T, PLCTimerSampleTime=0.001, PLCBlockType=TON, PLCPOUType=stdFB, PLCOperandAccess=ReadWrite, PLCOperandExpression=xxx_PLC_VAR_T}
      mask prompts: PLCOperandTag "Timer Tag:"; PLCTimerSampleTime "Timer Sample Time:"
      mask init:
      | block = gcb;
      | maskObj = Simulink.Mask.get(block);
      | maskObj.Display = sprintf('disp([''%s'' newline newline ''%s'']);', PLCBlockType, PLCOperandTag);
      | slplc.callbacks.initInstruction(block);
      settings: AttributesFormatString=%<PLCBlockType>: %<PLCOperandTag>
      mask Help: web([docroot '/plccoder/ref/ton' '.html']);
      mask DialogControl PLCBlockTitle Prompt: Timer On Delay (TON)
      mask Display: disp(['TON' newline newline 'T']);
  Up to Parent POU : Subsystem  DisableCoverage=on  TreatAsAtomicUnit=on  mask{PLCBlockType=OpenParentPOU}
      settings: OpenFcn=slplc.callbacks.openParentPOUBlock(gcb);
      mask Help: web([docroot '/plccoder/ref/uptoparentpou' '.html']);
      mask DialogControl PLCBlockTitle Prompt: Add Single Rung
  Variable Read : Subsystem  Priority=235  TreatAsAtomicUnit=on  mask{PLCOperandTag=VARVEL, PLCBlockType=VariableRead, PLCOperandAccess=Read, PLCPOUType=VariableRead, PLCOperandExpression=xxx_PLC_VAR_VARVEL}
      mask prompts: PLCOperandTag "Data Tag:"
      mask init:
      | block = gcb;
      | maskObj = Simulink.Mask.get(block);
      | maskObj.Display = sprintf('disp(''%s'');', PLCOperandTag);
      | slplc.callbacks.initInstruction(block);
      mask Help: web([docroot '/plccoder/ref/variableread' '.html']);
      mask DialogControl PLCBlockTitle Prompt: Data Tag Read
      mask Display: disp('VARVEL');
  Variable Read1 : Subsystem  Priority=84  TreatAsAtomicUnit=on  mask{PLCOperandTag=Floor_1, PLCBlockType=VariableRead, PLCOperandAccess=Read, PLCPOUType=VariableRead, PLCOperandExpression=xxx_PLC_VAR_Floor_1}
      mask prompts: PLCOperandTag "Data Tag:"
      mask init:
      | block = gcb;
      | maskObj = Simulink.Mask.get(block);
      | maskObj.Display = sprintf('disp(''%s'');', PLCOperandTag);
      | slplc.callbacks.initInstruction(block);
      mask Help: web([docroot '/plccoder/ref/variableread' '.html']);
      mask DialogControl PLCBlockTitle Prompt: Data Tag Read
      mask Display: disp('Floor_1');
  Variable Read10 : Subsystem  Priority=272  TreatAsAtomicUnit=on  mask{PLCOperandTag=VARVEL, PLCBlockType=VariableRead, PLCOperandAccess=Read, PLCPOUType=VariableRead, PLCOperandExpression=xxx_PLC_VAR_VARVEL}
      mask prompts: PLCOperandTag "Data Tag:"
      mask init:
      | block = gcb;
      | maskObj = Simulink.Mask.get(block);
      | maskObj.Display = sprintf('disp(''%s'');', PLCOperandTag);
      | slplc.callbacks.initInstruction(block);
      mask Help: web([docroot '/plccoder/ref/variableread' '.html']);
      mask DialogControl PLCBlockTitle Prompt: Data Tag Read
      mask Display: disp('VARVEL');
  Variable Read11 : Subsystem  Priority=286  TreatAsAtomicUnit=on  mask{PLCOperandTag=VARVEL, PLCBlockType=VariableRead, PLCOperandAccess=Read, PLCPOUType=VariableRead, PLCOperandExpression=xxx_PLC_VAR_VARVEL}
      mask prompts: PLCOperandTag "Data Tag:"
      mask init:
      | block = gcb;
      | maskObj = Simulink.Mask.get(block);
      | maskObj.Display = sprintf('disp(''%s'');', PLCOperandTag);
      | slplc.callbacks.initInstruction(block);
      mask Help: web([docroot '/plccoder/ref/variableread' '.html']);
      mask DialogControl PLCBlockTitle Prompt: Data Tag Read
      mask Display: disp('VARVEL');
  Variable Read12 : Subsystem  Priority=294  TreatAsAtomicUnit=on  mask{PLCOperandTag=VARVEL, PLCBlockType=VariableRead, PLCOperandAccess=Read, PLCPOUType=VariableRead, PLCOperandExpression=xxx_PLC_VAR_VARVEL}
      mask prompts: PLCOperandTag "Data Tag:"
      mask init:
      | block = gcb;
      | maskObj = Simulink.Mask.get(block);
      | maskObj.Display = sprintf('disp(''%s'');', PLCOperandTag);
      | slplc.callbacks.initInstruction(block);
      mask Help: web([docroot '/plccoder/ref/variableread' '.html']);
      mask DialogControl PLCBlockTitle Prompt: Data Tag Read
      mask Display: disp('VARVEL');
  Variable Read13 : Subsystem  Priority=265  TreatAsAtomicUnit=on  mask{PLCOperandTag=VARVEL, PLCBlockType=VariableRead, PLCOperandAccess=Read, PLCPOUType=VariableRead, PLCOperandExpression=xxx_PLC_VAR_VARVEL}
      mask prompts: PLCOperandTag "Data Tag:"
      mask init:
      | block = gcb;
      | maskObj = Simulink.Mask.get(block);
      | maskObj.Display = sprintf('disp(''%s'');', PLCOperandTag);
      | slplc.callbacks.initInstruction(block);
      mask Help: web([docroot '/plccoder/ref/variableread' '.html']);
      mask DialogControl PLCBlockTitle Prompt: Data Tag Read
      mask Display: disp('VARVEL');
  Variable Read14 : Subsystem  Priority=279  TreatAsAtomicUnit=on  mask{PLCOperandTag=VARVEL, PLCBlockType=VariableRead, PLCOperandAccess=Read, PLCPOUType=VariableRead, PLCOperandExpression=xxx_PLC_VAR_VARVEL}
      mask prompts: PLCOperandTag "Data Tag:"
      mask init:
      | block = gcb;
      | maskObj = Simulink.Mask.get(block);
      | maskObj.Display = sprintf('disp(''%s'');', PLCOperandTag);
      | slplc.callbacks.initInstruction(block);
      mask Help: web([docroot '/plccoder/ref/variableread' '.html']);
      mask DialogControl PLCBlockTitle Prompt: Data Tag Read
      mask Display: disp('VARVEL');
  Variable Read15 : Subsystem  Priority=300  TreatAsAtomicUnit=on  mask{PLCOperandTag=VARVEL, PLCBlockType=VariableRead, PLCOperandAccess=Read, PLCPOUType=VariableRead, PLCOperandExpression=xxx_PLC_VAR_VARVEL}
      mask prompts: PLCOperandTag "Data Tag:"
      mask init:
      | block = gcb;
      | maskObj = Simulink.Mask.get(block);
      | maskObj.Display = sprintf('disp(''%s'');', PLCOperandTag);
      | slplc.callbacks.initInstruction(block);
      mask Help: web([docroot '/plccoder/ref/variableread' '.html']);
      mask DialogControl PLCBlockTitle Prompt: Data Tag Read
      mask Display: disp('VARVEL');
  Variable Read16 : Subsystem  Priority=305  TreatAsAtomicUnit=on  mask{PLCOperandTag=Current_floor, PLCBlockType=VariableRead, PLCOperandAccess=Read, PLCPOUType=VariableRead, PLCOperandExpression=xxx_PLC_VAR_Current_floor}
      mask prompts: PLCOperandTag "Data Tag:"
      mask init:
      | block = gcb;
      | maskObj = Simulink.Mask.get(block);
      | maskObj.Display = sprintf('disp(''%s'');', PLCOperandTag);
      | slplc.callbacks.initInstruction(block);
      mask Help: web([docroot '/plccoder/ref/variableread' '.html']);
      mask DialogControl PLCBlockTitle Prompt: Data Tag Read
      mask Display: disp('Current_floor');
  Variable Read2 : Subsystem  Priority=77  TreatAsAtomicUnit=on  mask{PLCOperandTag=Floor_2, PLCBlockType=VariableRead, PLCOperandAccess=Read, PLCPOUType=VariableRead, PLCOperandExpression=xxx_PLC_VAR_Floor_2}
      mask prompts: PLCOperandTag "Data Tag:"
      mask init:
      | block = gcb;
      | maskObj = Simulink.Mask.get(block);
      | maskObj.Display = sprintf('disp(''%s'');', PLCOperandTag);
      | slplc.callbacks.initInstruction(block);
      mask Help: web([docroot '/plccoder/ref/variableread' '.html']);
      mask DialogControl PLCBlockTitle Prompt: Data Tag Read
      mask Display: disp('Floor_2');
  Variable Read3 : Subsystem  Priority=67  TreatAsAtomicUnit=on  mask{PLCOperandTag=Floor_3, PLCBlockType=VariableRead, PLCOperandAccess=Read, PLCPOUType=VariableRead, PLCOperandExpression=xxx_PLC_VAR_Floor_3}
      mask prompts: PLCOperandTag "Data Tag:"
      mask init:
      | block = gcb;
      | maskObj = Simulink.Mask.get(block);
      | maskObj.Display = sprintf('disp(''%s'');', PLCOperandTag);
      | slplc.callbacks.initInstruction(block);
      mask Help: web([docroot '/plccoder/ref/variableread' '.html']);
      mask DialogControl PLCBlockTitle Prompt: Data Tag Read
      mask Display: disp('Floor_3');
  Variable Read4 : Subsystem  Priority=107  TreatAsAtomicUnit=on  mask{PLCOperandTag=Floor_1, PLCBlockType=VariableRead, PLCOperandAccess=Read, PLCPOUType=VariableRead, PLCOperandExpression=xxx_PLC_VAR_Floor_1}
      mask prompts: PLCOperandTag "Data Tag:"
      mask init:
      | block = gcb;
      | maskObj = Simulink.Mask.get(block);
      | maskObj.Display = sprintf('disp(''%s'');', PLCOperandTag);
      | slplc.callbacks.initInstruction(block);
      mask Help: web([docroot '/plccoder/ref/variableread' '.html']);
      mask DialogControl PLCBlockTitle Prompt: Data Tag Read
      mask Display: disp('Floor_1');
  Variable Read5 : Subsystem  Priority=108  TreatAsAtomicUnit=on  mask{PLCOperandTag=Current_floor, PLCBlockType=VariableRead, PLCOperandAccess=Read, PLCPOUType=VariableRead, PLCOperandExpression=xxx_PLC_VAR_Current_floor}
      mask prompts: PLCOperandTag "Data Tag:"
      mask init:
      | block = gcb;
      | maskObj = Simulink.Mask.get(block);
      | maskObj.Display = sprintf('disp(''%s'');', PLCOperandTag);
      | slplc.callbacks.initInstruction(block);
      mask Help: web([docroot '/plccoder/ref/variableread' '.html']);
      mask DialogControl PLCBlockTitle Prompt: Data Tag Read
      mask Display: disp('Current_floor');
  Variable Read6 : Subsystem  Priority=99  TreatAsAtomicUnit=on  mask{PLCOperandTag=Floor_2, PLCBlockType=VariableRead, PLCOperandAccess=Read, PLCPOUType=VariableRead, PLCOperandExpression=xxx_PLC_VAR_Floor_2}
      mask prompts: PLCOperandTag "Data Tag:"
      mask init:
      | block = gcb;
      | maskObj = Simulink.Mask.get(block);
      | maskObj.Display = sprintf('disp(''%s'');', PLCOperandTag);
      | slplc.callbacks.initInstruction(block);
      mask Help: web([docroot '/plccoder/ref/variableread' '.html']);
      mask DialogControl PLCBlockTitle Prompt: Data Tag Read
      mask Display: disp('Floor_2');
  Variable Read7 : Subsystem  Priority=100  TreatAsAtomicUnit=on  mask{PLCOperandTag=Current_floor, PLCBlockType=VariableRead, PLCOperandAccess=Read, PLCPOUType=VariableRead, PLCOperandExpression=xxx_PLC_VAR_Current_floor}
      mask prompts: PLCOperandTag "Data Tag:"
      mask init:
      | block = gcb;
      | maskObj = Simulink.Mask.get(block);
      | maskObj.Display = sprintf('disp(''%s'');', PLCOperandTag);
      | slplc.callbacks.initInstruction(block);
      mask Help: web([docroot '/plccoder/ref/variableread' '.html']);
      mask DialogControl PLCBlockTitle Prompt: Data Tag Read
      mask Display: disp('Current_floor');
  Variable Read8 : Subsystem  Priority=91  TreatAsAtomicUnit=on  mask{PLCOperandTag=Floor_3, PLCBlockType=VariableRead, PLCOperandAccess=Read, PLCPOUType=VariableRead, PLCOperandExpression=xxx_PLC_VAR_Floor_3}
      mask prompts: PLCOperandTag "Data Tag:"
      mask init:
      | block = gcb;
      | maskObj = Simulink.Mask.get(block);
      | maskObj.Display = sprintf('disp(''%s'');', PLCOperandTag);
      | slplc.callbacks.initInstruction(block);
      mask Help: web([docroot '/plccoder/ref/variableread' '.html']);
      mask DialogControl PLCBlockTitle Prompt: Data Tag Read
      mask Display: disp('Floor_3');
  Variable Read9 : Subsystem  Priority=92  TreatAsAtomicUnit=on  mask{PLCOperandTag=Current_floor, PLCBlockType=VariableRead, PLCOperandAccess=Read, PLCPOUType=VariableRead, PLCOperandExpression=xxx_PLC_VAR_Current_floor}
      mask prompts: PLCOperandTag "Data Tag:"
      mask init:
      | block = gcb;
      | maskObj = Simulink.Mask.get(block);
      | maskObj.Display = sprintf('disp(''%s'');', PLCOperandTag);
      | slplc.callbacks.initInstruction(block);
      mask Help: web([docroot '/plccoder/ref/variableread' '.html']);
      mask DialogControl PLCBlockTitle Prompt: Data Tag Read
      mask Display: disp('Current_floor');
  Variable Write1 : Subsystem  Priority=86  TreatAsAtomicUnit=on  mask{PLCOperandTag=Current_floor, PLCBlockType=VariableWrite, PLCOperandAccess=Write, PLCPOUType=VariableWrite, PLCOperandExpression=xxx_PLC_VAR_Current_floor}
      mask prompts: PLCOperandTag "Data Tag:"
      mask init:
      | block = gcb;
      | maskObj = Simulink.Mask.get(block);
      | maskObj.Display = sprintf('disp(''%s'');', PLCOperandTag);
      | slplc.callbacks.initInstruction(block);
      | maskObj = Simulink.Mask.get(gcb);
      | maskObj.BlockDVGIcon = 'slplclib.VariableWrite';
      mask Help: web([docroot '/plccoder/ref/variablewrite' '.html']);
      mask DialogControl PLCBlockTitle Prompt: Data Tag Write
      mask Display: disp('Current_floor');
  Variable Write2 : Subsystem  Priority=79  TreatAsAtomicUnit=on  mask{PLCOperandTag=Current_floor, PLCBlockType=VariableWrite, PLCOperandAccess=Write, PLCPOUType=VariableWrite, PLCOperandExpression=xxx_PLC_VAR_Current_floor}
      mask prompts: PLCOperandTag "Data Tag:"
      mask init: same as elevator/PLCControllerSuite/__Logic/Task/Program/__Logic/Variable Write1
      mask Help: web([docroot '/plccoder/ref/variablewrite' '.html']);
      mask DialogControl PLCBlockTitle Prompt: Data Tag Write
      mask Display: disp('Current_floor');
  Variable Write3 : Subsystem  Priority=69  TreatAsAtomicUnit=on  mask{PLCOperandTag=Current_floor, PLCBlockType=VariableWrite, PLCOperandAccess=Write, PLCPOUType=VariableWrite, PLCOperandExpression=xxx_PLC_VAR_Current_floor}
      mask prompts: PLCOperandTag "Data Tag:"
      mask init: same as elevator/PLCControllerSuite/__Logic/Task/Program/__Logic/Variable Write1
      mask Help: web([docroot '/plccoder/ref/variablewrite' '.html']);
      mask DialogControl PLCBlockTitle Prompt: Data Tag Write
      mask Display: disp('Current_floor');
  Variable Write4 : Subsystem  Priority=275  TreatAsAtomicUnit=on  mask{PLCOperandTag=VARVEL, PLCBlockType=VariableWrite, PLCOperandAccess=Write, PLCPOUType=VariableWrite, PLCOperandExpression=xxx_PLC_VAR_VARVEL}
      mask prompts: PLCOperandTag "Data Tag:"
      mask init: same as elevator/PLCControllerSuite/__Logic/Task/Program/__Logic/Variable Write1
      mask Help: web([docroot '/plccoder/ref/variablewrite' '.html']);
      mask DialogControl PLCBlockTitle Prompt: Data Tag Write
      mask Display: disp('VARVEL');
  Variable Write5 : Subsystem  Priority=289  TreatAsAtomicUnit=on  mask{PLCOperandTag=VARVEL, PLCBlockType=VariableWrite, PLCOperandAccess=Write, PLCPOUType=VariableWrite, PLCOperandExpression=xxx_PLC_VAR_VARVEL}
      mask prompts: PLCOperandTag "Data Tag:"
      mask init: same as elevator/PLCControllerSuite/__Logic/Task/Program/__Logic/Variable Write1
      mask Help: web([docroot '/plccoder/ref/variablewrite' '.html']);
      mask DialogControl PLCBlockTitle Prompt: Data Tag Write
      mask Display: disp('VARVEL');
  Variable Write6 : Subsystem  Priority=297  TreatAsAtomicUnit=on  mask{PLCOperandTag=VARVEL, PLCBlockType=VariableWrite, PLCOperandAccess=Write, PLCPOUType=VariableWrite, PLCOperandExpression=xxx_PLC_VAR_VARVEL}
      mask prompts: PLCOperandTag "Data Tag:"
      mask init: same as elevator/PLCControllerSuite/__Logic/Task/Program/__Logic/Variable Write1
      mask Help: web([docroot '/plccoder/ref/variablewrite' '.html']);
      mask DialogControl PLCBlockTitle Prompt: Data Tag Write
      mask Display: disp('VARVEL');
  Variable Write7 : Subsystem  Priority=302  TreatAsAtomicUnit=on  mask{PLCOperandTag=VELOUT, PLCBlockType=VariableWrite, PLCOperandAccess=Write, PLCPOUType=VariableWrite, PLCOperandExpression=xxx_PLC_VAR_VELOUT}
      mask prompts: PLCOperandTag "Data Tag:"
      mask init: same as elevator/PLCControllerSuite/__Logic/Task/Program/__Logic/Variable Write1
      mask Help: web([docroot '/plccoder/ref/variablewrite' '.html']);
      mask DialogControl PLCBlockTitle Prompt: Data Tag Write
      mask Display: disp('VELOUT');
  Variable Write8 : Subsystem  Priority=307  TreatAsAtomicUnit=on  mask{PLCOperandTag=FLOOROUT, PLCBlockType=VariableWrite, PLCOperandAccess=Write, PLCPOUType=VariableWrite, PLCOperandExpression=xxx_PLC_VAR_FLOOROUT}
      mask prompts: PLCOperandTag "Data Tag:"
      mask init: same as elevator/PLCControllerSuite/__Logic/Task/Program/__Logic/Variable Write1
      mask Help: web([docroot '/plccoder/ref/variablewrite' '.html']);
      mask DialogControl PLCBlockTitle Prompt: Data Tag Write
      mask Display: disp('FLOOROUT');
  XIC : Subsystem  Priority=2  TreatAsAtomicUnit=on  mask{PLCOperandTag=Start, PLCBlockType=XIC, PLCPOUType=Contact, PLCOperandExpression=xxx_PLC_VAR_Start}
      mask prompts: PLCOperandTag "Operand Tag:"
      mask init:
      | slplc.callbacks.initInstruction(gcb);
      settings: AttributesFormatString=%<PLCOperandTag>
      mask Help: web([docroot '/plccoder/ref/xic' '.html']);
      mask DialogControl PLCBlockTitle Prompt: Examine If Closed (XIC)
  XIC1 : Subsystem  Priority=3  TreatAsAtomicUnit=on  mask{PLCOperandTag=StartHold, PLCBlockType=XIC, PLCPOUType=Contact, PLCOperandExpression=xxx_PLC_VAR_StartHold}
      mask prompts: PLCOperandTag "Operand Tag:"
      mask init:
      | slplc.callbacks.initInstruction(gcb);
      settings: AttributesFormatString=%<PLCOperandTag>
      mask Help: web([docroot '/plccoder/ref/xic' '.html']);
      mask DialogControl PLCBlockTitle Prompt: Examine If Closed (XIC)
  XIC10 : Subsystem  Priority=126  TreatAsAtomicUnit=on  mask{PLCOperandTag=StartHold, PLCBlockType=XIC, PLCPOUType=Contact, PLCOperandExpression=xxx_PLC_VAR_StartHold}
      mask prompts: PLCOperandTag "Operand Tag:"
      mask init:
      | slplc.callbacks.initInstruction(gcb);
      settings: AttributesFormatString=%<PLCOperandTag>
      mask Help: web([docroot '/plccoder/ref/xic' '.html']);
      mask DialogControl PLCBlockTitle Prompt: Examine If Closed (XIC)
  XIC100 : Subsystem  Priority=205  TreatAsAtomicUnit=on  mask{PLCOperandTag=GOINGDN, PLCBlockType=XIC, PLCPOUType=Contact, PLCOperandExpression=xxx_PLC_VAR_GOINGDN}
      mask prompts: PLCOperandTag "Operand Tag:"
      mask init:
      | slplc.callbacks.initInstruction(gcb);
      settings: AttributesFormatString=%<PLCOperandTag>
      mask Help: web([docroot '/plccoder/ref/xic' '.html']);
      mask DialogControl PLCBlockTitle Prompt: Examine If Closed (XIC)
  XIC101 : Subsystem  Priority=241  TreatAsAtomicUnit=on  mask{PLCOperandTag=StartHold, PLCBlockType=XIC, PLCPOUType=Contact, PLCOperandExpression=xxx_PLC_VAR_StartHold}
      mask prompts: PLCOperandTag "Operand Tag:"
      mask init:
      | slplc.callbacks.initInstruction(gcb);
      settings: AttributesFormatString=%<PLCOperandTag>
      mask Help: web([docroot '/plccoder/ref/xic' '.html']);
      mask DialogControl PLCBlockTitle Prompt: Examine If Closed (XIC)
  XIC102 : Subsystem  Priority=247  TreatAsAtomicUnit=on  mask{PLCOperandTag=StartHold, PLCBlockType=XIC, PLCPOUType=Contact, PLCOperandExpression=xxx_PLC_VAR_StartHold}
      mask prompts: PLCOperandTag "Operand Tag:"
      mask init:
      | slplc.callbacks.initInstruction(gcb);
      settings: AttributesFormatString=%<PLCOperandTag>
      mask Help: web([docroot '/plccoder/ref/xic' '.html']);
      mask DialogControl PLCBlockTitle Prompt: Examine If Closed (XIC)
  XIC103 : Subsystem  Priority=291  TreatAsAtomicUnit=on  mask{PLCOperandTag=StartHold, PLCBlockType=XIC, PLCPOUType=Contact, PLCOperandExpression=xxx_PLC_VAR_StartHold}
      mask prompts: PLCOperandTag "Operand Tag:"
      mask init:
      | slplc.callbacks.initInstruction(gcb);
      settings: AttributesFormatString=%<PLCOperandTag>
      mask Help: web([docroot '/plccoder/ref/xic' '.html']);
      mask DialogControl PLCBlockTitle Prompt: Examine If Closed (XIC)
  XIC104 : Subsystem  Priority=292  TreatAsAtomicUnit=on  mask{PLCOperandTag=RMPDN, PLCBlockType=XIC, PLCPOUType=Contact, PLCOperandExpression=xxx_PLC_VAR_RMPDN}
      mask prompts: PLCOperandTag "Operand Tag:"
      mask init:
      | slplc.callbacks.initInstruction(gcb);
      settings: AttributesFormatString=%<PLCOperandTag>
      mask Help: web([docroot '/plccoder/ref/xic' '.html']);
      mask DialogControl PLCBlockTitle Prompt: Examine If Closed (XIC)
  XIC105 : Subsystem  Priority=255  TreatAsAtomicUnit=on  mask{PLCOperandTag=StartHold, PLCBlockType=XIC, PLCPOUType=Contact, PLCOperandExpression=xxx_PLC_VAR_StartHold}
      mask prompts: PLCOperandTag "Operand Tag:"
      mask init:
      | slplc.callbacks.initInstruction(gcb);
      settings: AttributesFormatString=%<PLCOperandTag>
      mask Help: web([docroot '/plccoder/ref/xic' '.html']);
      mask DialogControl PLCBlockTitle Prompt: Examine If Closed (XIC)
  XIC106 : Subsystem  Priority=284  TreatAsAtomicUnit=on  mask{PLCOperandTag=StartHold, PLCBlockType=XIC, PLCPOUType=Contact, PLCOperandExpression=xxx_PLC_VAR_StartHold}
      mask prompts: PLCOperandTag "Operand Tag:"
      mask init:
      | slplc.callbacks.initInstruction(gcb);
      settings: AttributesFormatString=%<PLCOperandTag>
      mask Help: web([docroot '/plccoder/ref/xic' '.html']);
      mask DialogControl PLCBlockTitle Prompt: Examine If Closed (XIC)
  XIC107 : Subsystem  Priority=256  TreatAsAtomicUnit=on  mask{PLCOperandTag=MTRON, PLCBlockType=XIC, PLCPOUType=Contact, PLCOperandExpression=xxx_PLC_VAR_MTRON}
      mask prompts: PLCOperandTag "Operand Tag:"
      mask init:
      | slplc.callbacks.initInstruction(gcb);
      settings: AttributesFormatString=%<PLCOperandTag>
      mask Help: web([docroot '/plccoder/ref/xic' '.html']);
      mask DialogControl PLCBlockTitle Prompt: Examine If Closed (XIC)
  XIC108 : Subsystem  Priority=257  TreatAsAtomicUnit=on  mask{PLCOperandTag=RMPDNTRG, PLCBlockType=XIC, PLCPOUType=Contact, PLCOperandExpression=xxx_PLC_VAR_RMPDNTRG}
      mask prompts: PLCOperandTag "Operand Tag:"
      mask init:
      | slplc.callbacks.initInstruction(gcb);
      settings: AttributesFormatString=%<PLCOperandTag>
      mask Help: web([docroot '/plccoder/ref/xic' '.html']);
      mask DialogControl PLCBlockTitle Prompt: Examine If Closed (XIC)
  XIC109 : Subsystem  Priority=258  TreatAsAtomicUnit=on  mask{PLCOperandTag=RMPDN, PLCBlockType=XIC, PLCPOUType=Contact, PLCOperandExpression=xxx_PLC_VAR_RMPDN}
      mask prompts: PLCOperandTag "Operand Tag:"
      mask init:
      | slplc.callbacks.initInstruction(gcb);
      settings: AttributesFormatString=%<PLCOperandTag>
      mask Help: web([docroot '/plccoder/ref/xic' '.html']);
      mask DialogControl PLCBlockTitle Prompt: Examine If Closed (XIC)
  XIC11 : Subsystem  Priority=127  TreatAsAtomicUnit=on  mask{PLCOperandTag=F3PB, PLCBlockType=XIC, PLCPOUType=Contact, PLCOperandExpression=xxx_PLC_VAR_F3PB}
      mask prompts: PLCOperandTag "Operand Tag:"
      mask init:
      | slplc.callbacks.initInstruction(gcb);
      settings: AttributesFormatString=%<PLCOperandTag>
      mask Help: web([docroot '/plccoder/ref/xic' '.html']);
      mask DialogControl PLCBlockTitle Prompt: Examine If Closed (XIC)
  XIC110 : Subsystem  Priority=285  TreatAsAtomicUnit=on  mask{PLCOperandTag=DECSPD, PLCBlockType=XIC, PLCPOUType=Contact, PLCOperandExpression=xxx_PLC_VAR_DECSPD}
      mask prompts: PLCOperandTag "Operand Tag:"
      mask init:
      | slplc.callbacks.initInstruction(gcb);
      settings: AttributesFormatString=%<PLCOperandTag>
      mask Help: web([docroot '/plccoder/ref/xic' '.html']);
      mask DialogControl PLCBlockTitle Prompt: Examine If Closed (XIC)
  XIC111 : Subsystem  Priority=263  TreatAsAtomicUnit=on  mask{PLCOperandTag=StartHold, PLCBlockType=XIC, PLCPOUType=Contact, PLCOperandExpression=xxx_PLC_VAR_StartHold}
      mask prompts: PLCOperandTag "Operand Tag:"
      mask init:
      | slplc.callbacks.initInstruction(gcb);
      settings: AttributesFormatString=%<PLCOperandTag>
      mask Help: web([docroot '/plccoder/ref/xic' '.html']);
      mask DialogControl PLCBlockTitle Prompt: Examine If Closed (XIC)
  XIC112 : Subsystem  Priority=264  TreatAsAtomicUnit=on  mask{PLCOperandTag=RMPUP, PLCBlockType=XIC, PLCPOUType=Contact, PLCOperandExpression=xxx_PLC_VAR_RMPUP}
      mask prompts: PLCOperandTag "Operand Tag:"
      mask init:
      | slplc.callbacks.initInstruction(gcb);
      settings: AttributesFormatString=%<PLCOperandTag>
      mask Help: web([docroot '/plccoder/ref/xic' '.html']);
      mask DialogControl PLCBlockTitle Prompt: Examine If Closed (XIC)
  XIC113 : Subsystem  Priority=270  TreatAsAtomicUnit=on  mask{PLCOperandTag=StartHold, PLCBlockType=XIC, PLCPOUType=Contact, PLCOperandExpression=xxx_PLC_VAR_StartHold}
      mask prompts: PLCOperandTag "Operand Tag:"
      mask init:
      | slplc.callbacks.initInstruction(gcb);
      settings: AttributesFormatString=%<PLCOperandTag>
      mask Help: web([docroot '/plccoder/ref/xic' '.html']);
      mask DialogControl PLCBlockTitle Prompt: Examine If Closed (XIC)
  XIC114 : Subsystem  Priority=271  TreatAsAtomicUnit=on  mask{PLCOperandTag=INCSPD, PLCBlockType=XIC, PLCPOUType=Contact, PLCOperandExpression=xxx_PLC_VAR_INCSPD}
      mask prompts: PLCOperandTag "Operand Tag:"
      mask init:
      | slplc.callbacks.initInstruction(gcb);
      settings: AttributesFormatString=%<PLCOperandTag>
      mask Help: web([docroot '/plccoder/ref/xic' '.html']);
      mask DialogControl PLCBlockTitle Prompt: Examine If Closed (XIC)
  XIC115 : Subsystem  Priority=277  TreatAsAtomicUnit=on  mask{PLCOperandTag=StartHold, PLCBlockType=XIC, PLCPOUType=Contact, PLCOperandExpression=xxx_PLC_VAR_StartHold}
      mask prompts: PLCOperandTag "Operand Tag:"
      mask init:
      | slplc.callbacks.initInstruction(gcb);
      settings: AttributesFormatString=%<PLCOperandTag>
      mask Help: web([docroot '/plccoder/ref/xic' '.html']);
      mask DialogControl PLCBlockTitle Prompt: Examine If Closed (XIC)
  XIC116 : Subsystem  Priority=278  TreatAsAtomicUnit=on  mask{PLCOperandTag=RMPDN, PLCBlockType=XIC, PLCPOUType=Contact, PLCOperandExpression=xxx_PLC_VAR_RMPDN}
      mask prompts: PLCOperandTag "Operand Tag:"
      mask init:
      | slplc.callbacks.initInstruction(gcb);
      settings: AttributesFormatString=%<PLCOperandTag>
      mask Help: web([docroot '/plccoder/ref/xic' '.html']);
      mask DialogControl PLCBlockTitle Prompt: Examine If Closed (XIC)
  XIC117 : Subsystem  Priority=299  TreatAsAtomicUnit=on  mask{PLCOperandTag=StartHold, PLCBlockType=XIC, PLCPOUType=Contact, PLCOperandExpression=xxx_PLC_VAR_StartHold}
      mask prompts: PLCOperandTag "Operand Tag:"
      mask init:
      | slplc.callbacks.initInstruction(gcb);
      settings: AttributesFormatString=%<PLCOperandTag>
      mask Help: web([docroot '/plccoder/ref/xic' '.html']);
      mask DialogControl PLCBlockTitle Prompt: Examine If Closed (XIC)
  XIC118 : Subsystem  Priority=304  TreatAsAtomicUnit=on  mask{PLCOperandTag=StartHold, PLCBlockType=XIC, PLCPOUType=Contact, PLCOperandExpression=xxx_PLC_VAR_StartHold}
      mask prompts: PLCOperandTag "Operand Tag:"
      mask init:
      | slplc.callbacks.initInstruction(gcb);
      settings: AttributesFormatString=%<PLCOperandTag>
      mask Help: web([docroot '/plccoder/ref/xic' '.html']);
      mask DialogControl PLCBlockTitle Prompt: Examine If Closed (XIC)
  XIC12 : Subsystem  Priority=128  TreatAsAtomicUnit=on  mask{PLCOperandTag=F3PBHold, PLCBlockType=XIC, PLCPOUType=Contact, PLCOperandExpression=xxx_PLC_VAR_F3PBHold}
      mask prompts: PLCOperandTag "Operand Tag:"
      mask init:
      | slplc.callbacks.initInstruction(gcb);
      settings: AttributesFormatString=%<PLCOperandTag>
      mask Help: web([docroot '/plccoder/ref/xic' '.html']);
      mask DialogControl PLCBlockTitle Prompt: Examine If Closed (XIC)
  XIC13 : Subsystem  Priority=142  TreatAsAtomicUnit=on  mask{PLCOperandTag=F2DownB, PLCBlockType=XIC, PLCPOUType=Contact, PLCOperandExpression=xxx_PLC_VAR_F2DownB}
      mask prompts: PLCOperandTag "Operand Tag:"
      mask init:
      | slplc.callbacks.initInstruction(gcb);
      settings: AttributesFormatString=%<PLCOperandTag>
      mask Help: web([docroot '/plccoder/ref/xic' '.html']);
      mask DialogControl PLCBlockTitle Prompt: Examine If Closed (XIC)
  XIC14 : Subsystem  Priority=133  TreatAsAtomicUnit=on  mask{PLCOperandTag=StartHold, PLCBlockType=XIC, PLCPOUType=Contact, PLCOperandExpression=xxx_PLC_VAR_StartHold}
      mask prompts: PLCOperandTag "Operand Tag:"
      mask init:
      | slplc.callbacks.initInstruction(gcb);
      settings: AttributesFormatString=%<PLCOperandTag>
      mask Help: web([docroot '/plccoder/ref/xic' '.html']);
      mask DialogControl PLCBlockTitle Prompt: Examine If Closed (XIC)
  XIC15 : Subsystem  Priority=134  TreatAsAtomicUnit=on  mask{PLCOperandTag=F1UpB, PLCBlockType=XIC, PLCPOUType=Contact, PLCOperandExpression=xxx_PLC_VAR_F1UpB}
      mask prompts: PLCOperandTag "Operand Tag:"
      mask init:
      | slplc.callbacks.initInstruction(gcb);
      settings: AttributesFormatString=%<PLCOperandTag>
      mask Help: web([docroot '/plccoder/ref/xic' '.html']);
      mask DialogControl PLCBlockTitle Prompt: Examine If Closed (XIC)
  XIC16 : Subsystem  Priority=135  TreatAsAtomicUnit=on  mask{PLCOperandTag=F1UpBHold, PLCBlockType=XIC, PLCPOUType=Contact, PLCOperandExpression=xxx_PLC_VAR_F1UpBHold}
      mask prompts: PLCOperandTag "Operand Tag:"
      mask init:
      | slplc.callbacks.initInstruction(gcb);
      settings: AttributesFormatString=%<PLCOperandTag>
      mask Help: web([docroot '/plccoder/ref/xic' '.html']);
      mask DialogControl PLCBlockTitle Prompt: Examine If Closed (XIC)
  XIC17 : Subsystem  Priority=143  TreatAsAtomicUnit=on  mask{PLCOperandTag=F2UpDownBHold, PLCBlockType=XIC, PLCPOUType=Contact, PLCOperandExpression=xxx_PLC_VAR_F2UpDownBHold}
      mask prompts: PLCOperandTag "Operand Tag:"
      mask init:
      | slplc.callbacks.initInstruction(gcb);
      settings: AttributesFormatString=%<PLCOperandTag>
      mask Help: web([docroot '/plccoder/ref/xic' '.html']);
      mask DialogControl PLCBlockTitle Prompt: Examine If Closed (XIC)
  XIC18 : Subsystem  Priority=149  TreatAsAtomicUnit=on  mask{PLCOperandTag=StartHold, PLCBlockType=XIC, PLCPOUType=Contact, PLCOperandExpression=xxx_PLC_VAR_StartHold}
      mask prompts: PLCOperandTag "Operand Tag:"
      mask init:
      | slplc.callbacks.initInstruction(gcb);
      settings: AttributesFormatString=%<PLCOperandTag>
      mask Help: web([docroot '/plccoder/ref/xic' '.html']);
      mask DialogControl PLCBlockTitle Prompt: Examine If Closed (XIC)
  XIC19 : Subsystem  Priority=150  TreatAsAtomicUnit=on  mask{PLCOperandTag=F3DownB, PLCBlockType=XIC, PLCPOUType=Contact, PLCOperandExpression=xxx_PLC_VAR_F3DownB}
      mask prompts: PLCOperandTag "Operand Tag:"
      mask init:
      | slplc.callbacks.initInstruction(gcb);
      settings: AttributesFormatString=%<PLCOperandTag>
      mask Help: web([docroot '/plccoder/ref/xic' '.html']);
      mask DialogControl PLCBlockTitle Prompt: Examine If Closed (XIC)
  XIC2 : Subsystem  Priority=112  TreatAsAtomicUnit=on  mask{PLCOperandTag=StartHold, PLCBlockType=XIC, PLCPOUType=Contact, PLCOperandExpression=xxx_PLC_VAR_StartHold}
      mask prompts: PLCOperandTag "Operand Tag:"
      mask init:
      | slplc.callbacks.initInstruction(gcb);
      settings: AttributesFormatString=%<PLCOperandTag>
      mask Help: web([docroot '/plccoder/ref/xic' '.html']);
      mask DialogControl PLCBlockTitle Prompt: Examine If Closed (XIC)
  XIC20 : Subsystem  Priority=151  TreatAsAtomicUnit=on  mask{PLCOperandTag=F3DownBHold, PLCBlockType=XIC, PLCPOUType=Contact, PLCOperandExpression=xxx_PLC_VAR_F3DownBHold}
      mask prompts: PLCOperandTag "Operand Tag:"
      mask init:
      | slplc.callbacks.initInstruction(gcb);
      settings: AttributesFormatString=%<PLCOperandTag>
      mask Help: web([docroot '/plccoder/ref/xic' '.html']);
      mask DialogControl PLCBlockTitle Prompt: Examine If Closed (XIC)
  XIC21 : Subsystem  Priority=156  TreatAsAtomicUnit=on  mask{PLCOperandTag=StartHold, PLCBlockType=XIC, PLCPOUType=Contact, PLCOperandExpression=xxx_PLC_VAR_StartHold}
      mask prompts: PLCOperandTag "Operand Tag:"
      mask init:
      | slplc.callbacks.initInstruction(gcb);
      settings: AttributesFormatString=%<PLCOperandTag>
      mask Help: web([docroot '/plccoder/ref/xic' '.html']);
      mask DialogControl PLCBlockTitle Prompt: Examine If Closed (XIC)
  XIC22 : Subsystem  Priority=157  TreatAsAtomicUnit=on  mask{PLCOperandTag=F2UpDownBHold, PLCBlockType=XIC, PLCPOUType=Contact, PLCOperandExpression=xxx_PLC_VAR_F2UpDownBHold}
      mask prompts: PLCOperandTag "Operand Tag:"
      mask init:
      | slplc.callbacks.initInstruction(gcb);
      settings: AttributesFormatString=%<PLCOperandTag>
      mask Help: web([docroot '/plccoder/ref/xic' '.html']);
      mask DialogControl PLCBlockTitle Prompt: Examine If Closed (XIC)
  XIC23 : Subsystem  Priority=158  TreatAsAtomicUnit=on  mask{PLCOperandTag=F2PBHold, PLCBlockType=XIC, PLCPOUType=Contact, PLCOperandExpression=xxx_PLC_VAR_F2PBHold}
      mask prompts: PLCOperandTag "Operand Tag:"
      mask init:
      | slplc.callbacks.initInstruction(gcb);
      settings: AttributesFormatString=%<PLCOperandTag>
      mask Help: web([docroot '/plccoder/ref/xic' '.html']);
      mask DialogControl PLCBlockTitle Prompt: Examine If Closed (XIC)
  XIC24 : Subsystem  Priority=162  TreatAsAtomicUnit=on  mask{PLCOperandTag=F3DownBHold, PLCBlockType=XIC, PLCPOUType=Contact, PLCOperandExpression=xxx_PLC_VAR_F3DownBHold}
      mask prompts: PLCOperandTag "Operand Tag:"
      mask init:
      | slplc.callbacks.initInstruction(gcb);
      settings: AttributesFormatString=%<PLCOperandTag>
      mask Help: web([docroot '/plccoder/ref/xic' '.html']);
      mask DialogControl PLCBlockTitle Prompt: Examine If Closed (XIC)
  XIC25 : Subsystem  Priority=163  TreatAsAtomicUnit=on  mask{PLCOperandTag=F3PBHold, PLCBlockType=XIC, PLCPOUType=Contact, PLCOperandExpression=xxx_PLC_VAR_F3PBHold}
      mask prompts: PLCOperandTag "Operand Tag:"
      mask init:
      | slplc.callbacks.initInstruction(gcb);
      settings: AttributesFormatString=%<PLCOperandTag>
      mask Help: web([docroot '/plccoder/ref/xic' '.html']);
      mask DialogControl PLCBlockTitle Prompt: Examine If Closed (XIC)
  XIC26 : Subsystem  Priority=169  TreatAsAtomicUnit=on  mask{PLCOperandTag=StartHold, PLCBlockType=XIC, PLCPOUType=Contact, PLCOperandExpression=xxx_PLC_VAR_StartHold}
      mask prompts: PLCOperandTag "Operand Tag:"
      mask init:
      | slplc.callbacks.initInstruction(gcb);
      settings: AttributesFormatString=%<PLCOperandTag>
      mask Help: web([docroot '/plccoder/ref/xic' '.html']);
      mask DialogControl PLCBlockTitle Prompt: Examine If Closed (XIC)
  XIC27 : Subsystem  Priority=170  TreatAsAtomicUnit=on  mask{PLCOperandTag=F2UpDownBHold, PLCBlockType=XIC, PLCPOUType=Contact, PLCOperandExpression=xxx_PLC_VAR_F2UpDownBHold}
      mask prompts: PLCOperandTag "Operand Tag:"
      mask init:
      | slplc.callbacks.initInstruction(gcb);
      settings: AttributesFormatString=%<PLCOperandTag>
      mask Help: web([docroot '/plccoder/ref/xic' '.html']);
      mask DialogControl PLCBlockTitle Prompt: Examine If Closed (XIC)
  XIC28 : Subsystem  Priority=171  TreatAsAtomicUnit=on  mask{PLCOperandTag=F2PBHold, PLCBlockType=XIC, PLCPOUType=Contact, PLCOperandExpression=xxx_PLC_VAR_F2PBHold}
      mask prompts: PLCOperandTag "Operand Tag:"
      mask init:
      | slplc.callbacks.initInstruction(gcb);
      settings: AttributesFormatString=%<PLCOperandTag>
      mask Help: web([docroot '/plccoder/ref/xic' '.html']);
      mask DialogControl PLCBlockTitle Prompt: Examine If Closed (XIC)
  XIC29 : Subsystem  Priority=175  TreatAsAtomicUnit=on  mask{PLCOperandTag=F1UpBHold, PLCBlockType=XIC, PLCPOUType=Contact, PLCOperandExpression=xxx_PLC_VAR_F1UpBHold}
      mask prompts: PLCOperandTag "Operand Tag:"
      mask init:
      | slplc.callbacks.initInstruction(gcb);
      settings: AttributesFormatString=%<PLCOperandTag>
      mask Help: web([docroot '/plccoder/ref/xic' '.html']);
